simulink model "grid_nash"  (R2023b)
settings: Solver=ode23s  StartTime=0.0  StopTime=32  RelTol=1e-3
values from neighbouring files (symbols this model uses):
  lambda_compensator = -0.01    [model_parameters.m]
  nbus = 6    [model_parameters.m]
  Ts = 5e-6    (= 5e-06)    [model_parameters.m]
undefined symbols (not defined in the file or in its folder): AG, gcbh, Grid, IBR, L, SG, sps_rtmsupport, TX
libraries: spsThreePhaseVIMeasurementLib x13, spsFourierLib x13, spsPowerPositiveSequenceLib x13, spsThreePhaseSeriesRLCBranchLib x10, spsThreePhaseSeriesRLCLoadLib x10, spsThreePhaseTransformerTwoWindingsLib x10, spsDCVoltageSourceLib x8, spsFirstOrderFilterLib x8, spsabctodq0Lib x8, spsSimplifiedSynchronousMachinepuUnitsLib x6, spsGroundLib x4, spsUniversalBridgeLib x4
(part 1 of 2)
settings Model: SimulationMode=rapid-accelerator  Creator=psernatorre  LastModifiedBy=psernatorre
settings DataIOCC: InitialState=initial_data_nash.xFinal  LoadInitialState=on  SaveFinalState=on  SaveOperatingPoint=on
settings GRTTargetCC: RTWCAPISignals=on  RTWCAPIParams=on

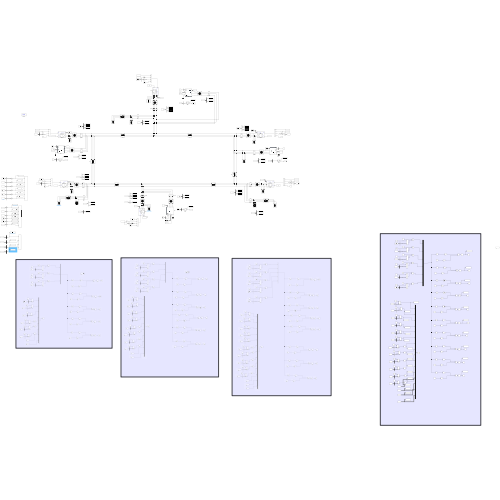
[thumbnail: Simulink's stored preview of the top-level diagram]
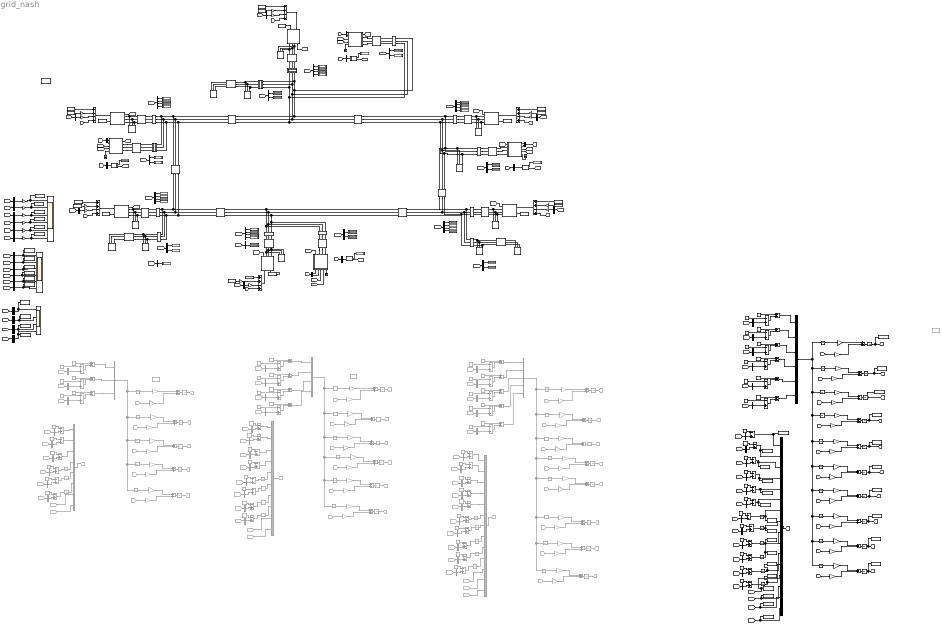
== system grid_nash ==
  note: NCG
  note: NCG
  note: NCG
  note: NCG
  Add{,6..7,20..22} (6 alike) : Sum  Inputs=++-+
  Add{1,3,14,23,25,27} (6 alike) : Sum  Inputs=+-
  Add{4..5,10,15,19,29..32,106} (10 alike) : Sum
  Add{39,44,51,56,61,68,73,78,83,90,95,100} (12 alike) : Sum  Commented=on  Inputs=+-
  Add{41..43,46..48,50,54..55,58..60,63..65,67,71..72,74..76,80..82,85..87,89,93..94,96..98,101..103} (36 alike) : Sum  Commented=on  Inputs=-+
  Add{40,45,49,52..53,57,62,66,69..70,77,79,84,88,91..92,99,104..105} (19 alike) : Sum  Commented=on
  Add{2,8..9,11..13,16..18,24,26,28,33..38} (18 alike) : Sum  Inputs=-+
  B1_IBR1 : Subsystem  mask{Sbase=Grid.Sbase, Vbase=Grid.Vbase, f=Grid.f, Ts=Ts, label=B1_IBR1, enable_power_calc=on}
      mask prompts: Sbase "Sbase (3-phase VA)"; Vbase "Vbase (L-L Vrms)"; f "Frequency (Hz)"; Ts "Sample time (s)"; label "Measure label"; enable_power_calc "Enable power calculation"
      mask init:
      | set_param([gcb '/signal'],'GotoTag', label)
      mask DialogControl DescGroupVar Prompt: Bus and measurements
      mask DialogControl Bus Prompt: Measure voltage, magnitude and phase, active power, reactive power
  B1_SG1 : Subsystem  mask{Sbase=Grid.Sbase, Vbase=Grid.Vbase, f=Grid.f, Ts=Ts, label=B1_SG1, enable_power_calc=on}
      mask prompts: Sbase "Sbase (3-phase VA)"; Vbase "Vbase (L-L Vrms)"; f "Frequency (Hz)"; Ts "Sample time (s)"; label "Measure label"; enable_power_calc "Enable power calculation"
      mask init:
      | set_param([gcb '/signal'],'GotoTag', label)
      mask DialogControl DescGroupVar Prompt: Bus and measurements
      mask DialogControl Bus Prompt: Measure voltage, magnitude and phase, active power, reactive power
  B5_L : Subsystem  mask{Sbase=Grid.Sbase, Vbase=Grid.Vbase, f=Grid.f, Ts=Ts, label=B5_L, enable_power_calc=on}
      mask prompts: Sbase "Sbase (3-phase VA)"; Vbase "Vbase (L-L Vrms)"; f "Frequency (Hz)"; Ts "Sample time (s)"; label "Measure label"; enable_power_calc "Enable power calculation"
      mask init:
      | set_param([gcb '/signal'],'GotoTag', label)
      mask DialogControl DescGroupVar Prompt: Bus and measurements
      mask DialogControl Bus Prompt: Measure voltage, magnitude and phase, active power, reactive power
  B5_SG6 : Subsystem  mask{Sbase=Grid.Sbase, Vbase=Grid.Vbase, f=Grid.f, Ts=Ts, label=B5_SG6, enable_power_calc=on}
      mask prompts: Sbase "Sbase (3-phase VA)"; Vbase "Vbase (L-L Vrms)"; f "Frequency (Hz)"; Ts "Sample time (s)"; label "Measure label"; enable_power_calc "Enable power calculation"
      mask init:
      | set_param([gcb '/signal'],'GotoTag', label)
      mask DialogControl DescGroupVar Prompt: Bus and measurements
      mask DialogControl Bus Prompt: Measure voltage, magnitude and phase, active power, reactive power
  B6_IBR3 : Subsystem  mask{Sbase=Grid.Sbase, Vbase=Grid.Vbase, f=Grid.f, Ts=Ts, label=B6_IBR3, enable_power_calc=on}
      mask prompts: Sbase "Sbase (3-phase VA)"; Vbase "Vbase (L-L Vrms)"; f "Frequency (Hz)"; Ts "Sample time (s)"; label "Measure label"; enable_power_calc "Enable power calculation"
      mask init:
      | set_param([gcb '/signal'],'GotoTag', label)
      mask DialogControl DescGroupVar Prompt: Bus and measurements
      mask DialogControl Bus Prompt: Measure voltage, magnitude and phase, active power, reactive power
  B6_SG5 : Subsystem  mask{Sbase=Grid.Sbase, Vbase=Grid.Vbase, f=Grid.f, Ts=Ts, label=B6_SG5, enable_power_calc=on}
      mask prompts: Sbase "Sbase (3-phase VA)"; Vbase "Vbase (L-L Vrms)"; f "Frequency (Hz)"; Ts "Sample time (s)"; label "Measure label"; enable_power_calc "Enable power calculation"
      mask init:
      | set_param([gcb '/signal'],'GotoTag', label)
      mask DialogControl DescGroupVar Prompt: Bus and measurements
      mask DialogControl Bus Prompt: Measure voltage, magnitude and phase, active power, reactive power
  B7_IBR4 : Subsystem  mask{Sbase=Grid.Sbase, Vbase=Grid.Vbase, f=Grid.f, Ts=Ts, label=B7_IBR4, enable_power_calc=on}
      mask prompts: Sbase "Sbase (3-phase VA)"; Vbase "Vbase (L-L Vrms)"; f "Frequency (Hz)"; Ts "Sample time (s)"; label "Measure label"; enable_power_calc "Enable power calculation"
      mask init:
      | set_param([gcb '/signal'],'GotoTag', label)
      mask DialogControl DescGroupVar Prompt: Bus and measurements
      mask DialogControl Bus Prompt: Measure voltage, magnitude and phase, active power, reactive power
  B7_L : Subsystem  mask{Sbase=Grid.Sbase, Vbase=Grid.Vbase, f=Grid.f, Ts=Ts, label=B7_L, enable_power_calc=on}
      mask prompts: Sbase "Sbase (3-phase VA)"; Vbase "Vbase (L-L Vrms)"; f "Frequency (Hz)"; Ts "Sample time (s)"; label "Measure label"; enable_power_calc "Enable power calculation"
      mask init:
      | set_param([gcb '/signal'],'GotoTag', label)
      mask DialogControl DescGroupVar Prompt: Bus and measurements
      mask DialogControl Bus Prompt: Measure voltage, magnitude and phase, active power, reactive power
  B7_SG4 : Subsystem  mask{Sbase=Grid.Sbase, Vbase=Grid.Vbase, f=Grid.f, Ts=Ts, label=B7_SG4, enable_power_calc=on}
      mask prompts: Sbase "Sbase (3-phase VA)"; Vbase "Vbase (L-L Vrms)"; f "Frequency (Hz)"; Ts "Sample time (s)"; label "Measure label"; enable_power_calc "Enable power calculation"
      mask init:
      | set_param([gcb '/signal'],'GotoTag', label)
      mask DialogControl DescGroupVar Prompt: Bus and measurements
      mask DialogControl Bus Prompt: Measure voltage, magnitude and phase, active power, reactive power
  B8_IBR2 : Subsystem  mask{Sbase=Grid.Sbase, Vbase=Grid.Vbase, f=Grid.f, Ts=Ts, label=B8_IBR2, enable_power_calc=on}
      mask prompts: Sbase "Sbase (3-phase VA)"; Vbase "Vbase (L-L Vrms)"; f "Frequency (Hz)"; Ts "Sample time (s)"; label "Measure label"; enable_power_calc "Enable power calculation"
      mask init:
      | set_param([gcb '/signal'],'GotoTag', label)
      mask DialogControl DescGroupVar Prompt: Bus and measurements
      mask DialogControl Bus Prompt: Measure voltage, magnitude and phase, active power, reactive power
  B8_SG3 : Subsystem  mask{Sbase=Grid.Sbase, Vbase=Grid.Vbase, f=Grid.f, Ts=Ts, label=B8_SG3, enable_power_calc=on}
      mask prompts: Sbase "Sbase (3-phase VA)"; Vbase "Vbase (L-L Vrms)"; f "Frequency (Hz)"; Ts "Sample time (s)"; label "Measure label"; enable_power_calc "Enable power calculation"
      mask init:
      | set_param([gcb '/signal'],'GotoTag', label)
      mask DialogControl DescGroupVar Prompt: Bus and measurements
      mask DialogControl Bus Prompt: Measure voltage, magnitude and phase, active power, reactive power
  B9_L : Subsystem  mask{Sbase=Grid.Sbase, Vbase=Grid.Vbase, f=Grid.f, Ts=Ts, label=B9_L, enable_power_calc=on}
      mask prompts: Sbase "Sbase (3-phase VA)"; Vbase "Vbase (L-L Vrms)"; f "Frequency (Hz)"; Ts "Sample time (s)"; label "Measure label"; enable_power_calc "Enable power calculation"
      mask init:
      | set_param([gcb '/signal'],'GotoTag', label)
      mask DialogControl DescGroupVar Prompt: Bus and measurements
      mask DialogControl Bus Prompt: Measure voltage, magnitude and phase, active power, reactive power
  B9_SG2 : Subsystem  mask{Sbase=Grid.Sbase, Vbase=Grid.Vbase, f=Grid.f, Ts=Ts, label=B9_SG2, enable_power_calc=on}
      mask prompts: Sbase "Sbase (3-phase VA)"; Vbase "Vbase (L-L Vrms)"; f "Frequency (Hz)"; Ts "Sample time (s)"; label "Measure label"; enable_power_calc "Enable power calculation"
      mask init:
      | set_param([gcb '/signal'],'GotoTag', label)
      mask DialogControl DescGroupVar Prompt: Bus and measurements
      mask DialogControl Bus Prompt: Measure voltage, magnitude and phase, active power, reactive power
  Bus Selector{1,29,31,33,91..92} (6 alike) : BusSelector  OutputSignals=P,Q,Vmag,Vphase
  Bus Selector{8,10..11,19,32,42..45,95} (10 alike) : BusSelector  OutputSignals=P
  Bus Selector{3..7,9,12..13,16..18,20..22,24..25,28,30,34,37,39..41,46..54} (32 alike) : BusSelector  OutputSignals=Rotor speed wm (pu)
  Bus Selector{14..15,35,93} (4 alike) : BusSelector  OutputSignals=V
  Bus Selector{2,23,26..27,36,38,94} (7 alike) : BusSelector  OutputSignals=P,Q
  Bus Selector{55..90} (36 alike) : BusSelector  Commented=on  OutputSignals=Rotor speed wm (pu)
  Constant{,17,20,23..24,28} (6 alike) : Constant  Value=1.02
  Constant1 : Constant  Value=0.20
  Constant{2,4,6..7,9..14,16,18..19,22,27,30,32,34,36..41} (24 alike) : Constant
  Constant15 : Constant  Value=0.10
  Constant21 : Constant  Value=0.05
  Constant25 : Constant  Value=0.50
  Constant26 : Constant  Value=0.40
  Constant29 : Constant  Value=0.05
  Constant{3,5,8,31,33,35} (6 alike) : Constant  Value=0
  Constant{42..46,48,50..51,53..58,60,62..63,65..66,68..74,76,78..79,81..82,84..86,88..89} (36 alike) : Constant  Commented=on
  Constant{47,49,52,59,61,64,67,75,77,80,83,87} (12 alike) : Constant  Commented=on  Value=0
  Demux{1..4} (4 alike) : Demux  Outputs=2
  Display{1..44} (44 alike) : Display
      settings: Format=bank
  From{84,88,92,100,104,108,117,121,125} (9 alike) : From  Commented=on  GotoTag=m_SG2
  From{85,91,93,101,107,109,118,124,126} (9 alike) : From  Commented=on  GotoTag=m_SG3
  From{83,86..87,99,102..103,119..120,136} (9 alike) : From  Commented=on  GotoTag=m_SG1
  From{81,89..90,94..95,97,105..106,110..111,116,122..123,127..128,133..134,141..142} (19 alike) : From  Commented=on
  From112 : From  Commented=on  GotoTag=m_IBR2
  From{113..115,130..132} (6 alike) : From  Commented=on  GotoTag=m_SG4
  From{6,12,24,26,34..35,70..72,150} (10 alike) : From
  From129 : From  Commented=on  GotoTag=m_IBR2
  From135 : From  Commented=on  GotoTag=m_IBR1
  From137 : From  Commented=on  GotoTag=m_SG5
  From138 : From  Commented=on  GotoTag=m_SG5
  From139 : From  Commented=on  GotoTag=m_SG5
  From140 : From  Commented=on  GotoTag=m_IBR3
  From82 : From  Commented=on  GotoTag=m_IBR1
  From96 : From  Commented=on  GotoTag=m_IBR2
  From98 : From  Commented=on  GotoTag=m_IBR1
  Gain{1,10..11,26..28} (6 alike) : Gain  Gain=Grid.f
  Gain12 : Gain  Gain=1/SG(4).Rp
  Gain13 : Gain  Gain=AG(4).Ki  Multiplication=Matrix(K*u)
  Gain14 : Gain  Gain=AG(4).Kp  Multiplication=Matrix(K*u)
  Gain15 : Gain  Gain=AG(5).Ki  Multiplication=Matrix(K*u)
  Gain16 : Gain  Gain=AG(5).Kp  Multiplication=Matrix(K*u)
  Gain17 : Gain  Gain=1/SG(2).Rp
  Gain18 : Gain  Gain=1/SG(2).Rp
  Gain19 : Gain  Gain=1/SG(3).Rp
  Gain2 : Gain  Gain=1/SG(1).Rp
  Gain20 : Gain  Gain=1/SG(3).Rp
  Gain21 : Gain  Gain=1/SG(4).Rp
  Gain22 : Gain  Gain=1/SG(5).Rp
  Gain23 : Gain  Gain=1/SG(5).Rp
  Gain24 : Gain  Gain=1/SG(6).Rp
  Gain25 : Gain  Gain=1/SG(6).Rp
  Gain29 : Gain  Gain=AG(6).Ki  Multiplication=Matrix(K*u)
  Gain3 : Gain  Gain=1/SG(1).Rp
  Gain30 : Gain  Gain=AG(6).Kp  Multiplication=Matrix(K*u)
  Gain31 : Gain  Gain=AG(7).Ki  Multiplication=Matrix(K*u)
  Gain32 : Gain  Gain=AG(7).Kp  Multiplication=Matrix(K*u)
  Gain33 : Gain  Gain=AG(8).Ki  Multiplication=Matrix(K*u)
  Gain34 : Gain  Gain=AG(8).Kp  Multiplication=Matrix(K*u)
  Gain35 : Gain  Gain=AG(9).Ki  Multiplication=Matrix(K*u)
  Gain36 : Gain  Gain=AG(9).Kp  Multiplication=Matrix(K*u)
  Gain37 : Gain  Commented=on  Gain=AG(4).Ki  Multiplication=Matrix(K*u)
  Gain38 : Gain  Commented=on  Gain=AG(4).Kp  Multiplication=Matrix(K*u)
  Gain39 : Gain  Commented=on  Gain=AG(5).Ki  Multiplication=Matrix(K*u)
  Gain4 : Gain  Gain=AG(1).Kp  Multiplication=Matrix(K*u)
  Gain40 : Gain  Commented=on  Gain=AG(5).Kp  Multiplication=Matrix(K*u)
  Gain41 : Gain  Commented=on  Gain=AG(1).Kp  Multiplication=Matrix(K*u)
  Gain42 : Gain  Commented=on  Gain=AG(1).Ki  Multiplication=Matrix(K*u)
  Gain43 : Gain  Commented=on  Gain=AG(2).Ki  Multiplication=Matrix(K*u)
  Gain44 : Gain  Commented=on  Gain=AG(2).Kp  Multiplication=Matrix(K*u)
  Gain45 : Gain  Commented=on  Gain=AG(3).Ki  Multiplication=Matrix(K*u)
  Gain46 : Gain  Commented=on  Gain=AG(3).Kp  Multiplication=Matrix(K*u)
  Gain47 : Gain  Commented=on  Gain=AG(5).Ki  Multiplication=Matrix(K*u)
  Gain48 : Gain  Commented=on  Gain=AG(5).Kp  Multiplication=Matrix(K*u)
  Gain49 : Gain  Commented=on  Gain=AG(6).Ki  Multiplication=Matrix(K*u)
  Gain5 : Gain  Gain=AG(1).Ki  Multiplication=Matrix(K*u)
  Gain50 : Gain  Commented=on  Gain=AG(6).Kp  Multiplication=Matrix(K*u)
  Gain51 : Gain  Commented=on  Gain=AG(1).Kp  Multiplication=Matrix(K*u)
  Gain52 : Gain  Commented=on  Gain=AG(1).Ki  Multiplication=Matrix(K*u)
  Gain53 : Gain  Commented=on  Gain=AG(2).Ki  Multiplication=Matrix(K*u)
  Gain54 : Gain  Commented=on  Gain=AG(2).Kp  Multiplication=Matrix(K*u)
  Gain55 : Gain  Commented=on  Gain=AG(3).Ki  Multiplication=Matrix(K*u)
  Gain56 : Gain  Commented=on  Gain=AG(3).Kp  Multiplication=Matrix(K*u)
  Gain57 : Gain  Commented=on  Gain=AG(4).Ki  Multiplication=Matrix(K*u)
  Gain58 : Gain  Commented=on  Gain=AG(4).Kp  Multiplication=Matrix(K*u)
  Gain59 : Gain  Commented=on  Gain=AG(6).Ki  Multiplication=Matrix(K*u)
  Gain6 : Gain  Gain=AG(2).Ki  Multiplication=Matrix(K*u)
  Gain60 : Gain  Commented=on  Gain=AG(6).Kp  Multiplication=Matrix(K*u)
  Gain61 : Gain  Commented=on  Gain=AG(7).Ki  Multiplication=Matrix(K*u)
  Gain62 : Gain  Commented=on  Gain=AG(7).Kp  Multiplication=Matrix(K*u)
  Gain63 : Gain  Commented=on  Gain=AG(1).Kp  Multiplication=Matrix(K*u)
  Gain64 : Gain  Commented=on  Gain=AG(1).Ki  Multiplication=Matrix(K*u)
  Gain65 : Gain  Commented=on  Gain=AG(2).Ki  Multiplication=Matrix(K*u)
  Gain66 : Gain  Commented=on  Gain=AG(2).Kp  Multiplication=Matrix(K*u)
  Gain67 : Gain  Commented=on  Gain=AG(3).Ki  Multiplication=Matrix(K*u)
  Gain68 : Gain  Commented=on  Gain=AG(3).Kp  Multiplication=Matrix(K*u)
  Gain69 : Gain  Commented=on  Gain=AG(4).Ki  Multiplication=Matrix(K*u)
  Gain7 : Gain  Gain=AG(2).Kp  Multiplication=Matrix(K*u)
  Gain70 : Gain  Commented=on  Gain=AG(4).Kp  Multiplication=Matrix(K*u)
  Gain71 : Gain  Commented=on  Gain=AG(5).Ki  Multiplication=Matrix(K*u)
  Gain72 : Gain  Commented=on  Gain=AG(5).Kp  Multiplication=Matrix(K*u)
  Gain73 : Gain  Commented=on  Gain=AG(8).Ki  Multiplication=Matrix(K*u)
  Gain74 : Gain  Commented=on  Gain=AG(8).Kp  Multiplication=Matrix(K*u)
  Gain75 : Gain  Gain=AG(10).Ki  Multiplication=Matrix(K*u)
  Gain76 : Gain  Gain=AG(10).Kp  Multiplication=Matrix(K*u)
  Gain8 : Gain  Gain=AG(3).Ki  Multiplication=Matrix(K*u)
  Gain9 : Gain  Gain=AG(3).Kp  Multiplication=Matrix(K*u)
  Goto2 : Goto
  Goto23 : Goto  Commented=on  GotoTag=u3
  Goto24 : Goto  Commented=on
  Goto25 : Goto  Commented=on  GotoTag=u7
  Goto26 : Goto  Commented=on  GotoTag=u8
  Goto27 : Goto  Commented=on  GotoTag=u1
  Goto28 : Goto  Commented=on  GotoTag=u2
  Goto29 : Goto  Commented=on  GotoTag=u3
  Goto30 : Goto  Commented=on
  Goto31 : Goto  Commented=on  GotoTag=u7
  Goto32 : Goto  Commented=on  GotoTag=u8
  Goto33 : Goto  Commented=on  GotoTag=u1
  Goto34 : Goto  Commented=on  GotoTag=u2
  Goto35 : Goto  Commented=on  GotoTag=u4
  Goto36 : Goto  Commented=on  GotoTag=u3
  Goto37 : Goto  Commented=on
  Goto38 : Goto  Commented=on  GotoTag=u7
  Goto39 : Goto  Commented=on  GotoTag=u8
  Goto40 : Goto  Commented=on  GotoTag=u1
  Goto41 : Goto  Commented=on  GotoTag=u2
  Goto42 : Goto  Commented=on  GotoTag=u4
  Goto43 : Goto  Commented=on  GotoTag=u5
  Goto44 : Goto  Commented=on  GotoTag=u9
  Ground{1..4} (4 alike) : spsGroundLib/Ground  LConnTagsString=a
  IBR1 : Subsystem  mask{S=Grid.Sbase, V=IBR(1).Vbase, Vdc=IBR(1).Vdc, Rf=IBR(1).Rf, Lf=IBR(1).Lf, Rc=IBR(1).Rc, Lc=IBR(1).Lc, Kp=IBR(1).Kp, Ki=IBR(1).Ki, f=Grid.f, Tf=IBR(1).Tf, Ts=Ts, enable_state_estimation=off, A_est=0, B_est=0, C_est=0, D_est=0}
      mask prompts: S "Pnom (VA)"; V "Vnom (Line Vrms)"; Vdc "Vdc (V)"; Rf "Rf (p.u.)"; Lf "Lf (p.u.)"; Rc "Rc (p.u.)"; Lc "Lc (p.u.)"; f "Frequency (Hz)"; Tf "Tf (feed-forward)"; Ts "Sample time (s)"; enable_state_estimation "Enable state estimation"
      mask DialogControl DescGroupVar Prompt: PLL-based grid-following IBR with LC filter
      mask DialogControl DescTextVar Prompt: Implements a grid-following inverter with LC filter with PI controllers in dq0-synchronous frames. It considers feed-forward compensation with first-order low-pass filter. Rf and Lf are impendances of the internal filter, and Rc and Lc are the impendances including a step-up transformer if there exists.
      mask Display: image('GFL_LC.png');
  IBR2 : Subsystem  mask{S=Grid.Sbase, V=IBR(2).Vbase, Vdc=IBR(2).Vdc, Rf=IBR(2).Rf, Lf=IBR(2).Lf, Rc=IBR(2).Rc, Lc=IBR(2).Lc, Kp=IBR(2).Kp, Ki=IBR(2).Ki, f=Grid.f, Tf=IBR(2).Tf, Ts=Ts, enable_state_estimation=off, A_est=0, B_est=0, C_est=0, D_est=0}
      mask prompts: S "Pnom (VA)"; V "Vnom (Line Vrms)"; Vdc "Vdc (V)"; Rf "Rf (p.u.)"; Lf "Lf (p.u.)"; Rc "Rc (p.u.)"; Lc "Lc (p.u.)"; f "Frequency (Hz)"; Tf "Tf (feed-forward)"; Ts "Sample time (s)"; enable_state_estimation "Enable state estimation"
      mask DialogControl DescGroupVar Prompt: PLL-based grid-following IBR with LC filter
      mask DialogControl DescTextVar Prompt: Implements a grid-following inverter with LC filter with PI controllers in dq0-synchronous frames. It considers feed-forward compensation with first-order low-pass filter. Rf and Lf are impendances of the internal filter, and Rc and Lc are the impendances including a step-up transformer if there exists.
      mask Display: image('GFL_LC.png');
  IBR3 : Subsystem  mask{S=Grid.Sbase, V=IBR(3).Vbase, Vdc=IBR(3).Vdc, Rf=IBR(3).Rf, Lf=IBR(3).Lf, Rc=IBR(3).Rc, Lc=IBR(3).Lc, Kp=IBR(3).Kp, Ki=IBR(3).Ki, f=Grid.f, Tf=IBR(3).Tf, Ts=Ts, enable_state_estimation=off, A_est=0, B_est=0, C_est=0, D_est=0}
      mask prompts: S "Pnom (VA)"; V "Vnom (Line Vrms)"; Vdc "Vdc (V)"; Rf "Rf (p.u.)"; Lf "Lf (p.u.)"; Rc "Rc (p.u.)"; Lc "Lc (p.u.)"; f "Frequency (Hz)"; Tf "Tf (feed-forward)"; Ts "Sample time (s)"; enable_state_estimation "Enable state estimation"
      mask DialogControl DescGroupVar Prompt: PLL-based grid-following IBR with LC filter
      mask DialogControl DescTextVar Prompt: Implements a grid-following inverter with LC filter with PI controllers in dq0-synchronous frames. It considers feed-forward compensation with first-order low-pass filter. Rf and Lf are impendances of the internal filter, and Rc and Lc are the impendances including a step-up transformer if there exists.
      mask Display: image('GFL_LC.png');
  IBR4 : Subsystem  mask{S=Grid.Sbase, V=IBR(2).Vbase, Vdc=IBR(2).Vdc, Rf=IBR(2).Rf, Lf=IBR(2).Lf, Rc=IBR(2).Rc, Lc=IBR(2).Lc, Kp=IBR(2).Kp, Ki=IBR(2).Ki, f=Grid.f, Tf=IBR(2).Tf, Ts=Ts, enable_state_estimation=off, A_est=0, B_est=0, C_est=0, D_est=0}
      mask prompts: S "Pnom (VA)"; V "Vnom (Line Vrms)"; Vdc "Vdc (V)"; Rf "Rf (p.u.)"; Lf "Lf (p.u.)"; Rc "Rc (p.u.)"; Lc "Lc (p.u.)"; f "Frequency (Hz)"; Tf "Tf (feed-forward)"; Ts "Sample time (s)"; enable_state_estimation "Enable state estimation"
      mask DialogControl DescGroupVar Prompt: PLL-based grid-following IBR with LC filter
      mask DialogControl DescTextVar Prompt: Implements a grid-following inverter with LC filter with PI controllers in dq0-synchronous frames. It considers feed-forward compensation with first-order low-pass filter. Rf and Lf are impendances of the internal filter, and Rc and Lc are the impendances including a step-up transformer if there exists.
      mask Display: image('GFL_LC.png');
  Integrator{,1..14,46} (16 alike) : Integrator
  Integrator{15..45} (31 alike) : Integrator  Commented=on
  Mux : Mux  Inputs=6
  Mux1 : Mux  Commented=on  Inputs=3
  Mux2 : Mux  Commented=on  Inputs=8
  Mux3 : Mux  Commented=on
  Mux4 : Mux  Commented=on  Inputs=10
  Mux5 : Mux  Commented=on  Inputs=5
  Mux6 : Mux  Inputs=16
  Mux7 : Mux  Commented=on  Inputs=13
  PLL (3ph) : Subsystem  AncestorBlock=|  DialogController=POWERSYS.PowerSysDialog  LoadFcn=sps_rtmsupport('LoadFcn', gcbh);  StartFcn=sps_rtmsupport('StartFcn', gcbh);  StopFcn=sps_rtmsupport('StopFcn', gcbh);  mask(PLL (3ph)){Fmin=45, Par_Init=[0, 60], ParK=[180, 3200, 1], TcD=1e-4, MaxRateChangeFreq=12, FilterCutOffFreq=25, Ts=Ts, AGC=on}
      | sps_lib/Control/PLL
      | (3ph)
      mask prompts: Fmin "Minimum frequency (Hz):"; Par_Init "Initial inputs [ Phase (degrees), Frequency (Hz) ]:"; ParK "Regulator gains [ Kp, Ki, Kd ]:"; TcD "Time constant for derivative action (s):"; MaxRateChangeFreq "Maximum rate of change of frequency (Hz/s):"; FilterCutOffFreq "Filter cut-off frequency for frequency measurement (Hz):"; Ts "Sample time:"; AGC "Enable automatic gain control"
      mask help:
      | This Phase Locked Loop (PLL) system can be used  to synchronize on a set of variable frequency, three-phase sinusoidal signals. If the Automatic Gain Control is enabled, the input (phase error) of the PLL regulator is scaled according to the input signals magnitude.
      |
      | For optimal performance, set regulator gains [ Kp Ki  Kd ] = [ 180  3200  1 ] and check the Enable Automatic Gain Control parameter.
      |
      | Input : Vector containing the normalized three-phase signals [Va Vb Vc]
      | Output 1:  Measured frequency (Hz) = w/(2pi)
      | Output 2:  Ramp w.t varying between  0 and 2*pi, synchronized on zero crossings of the fundamental (positive-sequence) of phase A.
      mask init:
      | block=gcb;
      | [WantBlockChoice,Ts,sps] = powericon('PLL3phInit',block,Fmin,Par_Init,ParK,TcD, MaxRateChangeFreq, FilterCutOffFreq, AGC,Ts);
      | powericon('SetInternalModels','set',block,WantBlockChoice);
      settings: CopyFcn=sps_rtmsupport('CopyFcn', gcbh);  DeleteFcn=sps_rtmsupport('DeleteFcn', gcbh);  UndoDeleteFcn=sps_rtmsupport('UndoDeleteFcn', gcbh);  ModelCloseFcn=sps_rtmsupport('ModelCloseFcn', gcbh);  PreSaveFcn=sps_rtmsupport('PreSaveFcn', gcbh);  PostSaveFcn=sps_rtmsupport('PostSaveFcn', gcbh);  NameChangeFcn=sps_rtmsupport('NameChangeFcn', gcbh);  PreCopyFcn=sps_rtmsupport('PreCopyFcn', gcbh);  OpenFcn=sps_rtmsupport('OpenFcn', gcbh, [8]);  CloseFcn=sps_rtmsupport('CloseFcn', gcbh);  PreDeleteFcn=sps_rtmsupport('PreDeleteFcn', gcbh);
      settings: LibrarySourceBlock=|
      | sps_lib/Control/PLL
      | (3ph)
      mask Help: helpview(psbhelp);
  PLL (3ph)1 : Subsystem  AncestorBlock=|  DialogController=POWERSYS.PowerSysDialog  LoadFcn=sps_rtmsupport('LoadFcn', gcbh);  StartFcn=sps_rtmsupport('StartFcn', gcbh);  StopFcn=sps_rtmsupport('StopFcn', gcbh);  mask(PLL (3ph)){Fmin=45, Par_Init=[0, 60], ParK=[180, 3200, 1], TcD=1e-4, MaxRateChangeFreq=12, FilterCutOffFreq=25, Ts=Ts, AGC=on}
      | sps_lib/Control/PLL
      | (3ph)
      mask prompts: Fmin "Minimum frequency (Hz):"; Par_Init "Initial inputs [ Phase (degrees), Frequency (Hz) ]:"; ParK "Regulator gains [ Kp, Ki, Kd ]:"; TcD "Time constant for derivative action (s):"; MaxRateChangeFreq "Maximum rate of change of frequency (Hz/s):"; FilterCutOffFreq "Filter cut-off frequency for frequency measurement (Hz):"; Ts "Sample time:"; AGC "Enable automatic gain control"
      mask help:
      | This Phase Locked Loop (PLL) system can be used  to synchronize on a set of variable frequency, three-phase sinusoidal signals. If the Automatic Gain Control is enabled, the input (phase error) of the PLL regulator is scaled according to the input signals magnitude.
      |
      | For optimal performance, set regulator gains [ Kp Ki  Kd ] = [ 180  3200  1 ] and check the Enable Automatic Gain Control parameter.
      |
      | Input : Vector containing the normalized three-phase signals [Va Vb Vc]
      | Output 1:  Measured frequency (Hz) = w/(2pi)
      | Output 2:  Ramp w.t varying between  0 and 2*pi, synchronized on zero crossings of the fundamental (positive-sequence) of phase A.
      mask init:
      | block=gcb;
      | [WantBlockChoice,Ts,sps] = powericon('PLL3phInit',block,Fmin,Par_Init,ParK,TcD, MaxRateChangeFreq, FilterCutOffFreq, AGC,Ts);
      | powericon('SetInternalModels','set',block,WantBlockChoice);
      settings: CopyFcn=sps_rtmsupport('CopyFcn', gcbh);  DeleteFcn=sps_rtmsupport('DeleteFcn', gcbh);  UndoDeleteFcn=sps_rtmsupport('UndoDeleteFcn', gcbh);  ModelCloseFcn=sps_rtmsupport('ModelCloseFcn', gcbh);  PreSaveFcn=sps_rtmsupport('PreSaveFcn', gcbh);  PostSaveFcn=sps_rtmsupport('PostSaveFcn', gcbh);  NameChangeFcn=sps_rtmsupport('NameChangeFcn', gcbh);  PreCopyFcn=sps_rtmsupport('PreCopyFcn', gcbh);  OpenFcn=sps_rtmsupport('OpenFcn', gcbh, [8]);  CloseFcn=sps_rtmsupport('CloseFcn', gcbh);  PreDeleteFcn=sps_rtmsupport('PreDeleteFcn', gcbh);
      settings: LibrarySourceBlock=|
      | sps_lib/Control/PLL
      | (3ph)
      mask Help: helpview(psbhelp);
  PLL (3ph)2 : Subsystem  AncestorBlock=|  DialogController=POWERSYS.PowerSysDialog  LoadFcn=sps_rtmsupport('LoadFcn', gcbh);  StartFcn=sps_rtmsupport('StartFcn', gcbh);  StopFcn=sps_rtmsupport('StopFcn', gcbh);  mask(PLL (3ph)){Fmin=45, Par_Init=[0, 60], ParK=[180, 3200, 1], TcD=1e-4, MaxRateChangeFreq=12, FilterCutOffFreq=25, Ts=Ts, AGC=on}
      | sps_lib/Control/PLL
      | (3ph)
      mask prompts: Fmin "Minimum frequency (Hz):"; Par_Init "Initial inputs [ Phase (degrees), Frequency (Hz) ]:"; ParK "Regulator gains [ Kp, Ki, Kd ]:"; TcD "Time constant for derivative action (s):"; MaxRateChangeFreq "Maximum rate of change of frequency (Hz/s):"; FilterCutOffFreq "Filter cut-off frequency for frequency measurement (Hz):"; Ts "Sample time:"; AGC "Enable automatic gain control"
      mask help:
      | This Phase Locked Loop (PLL) system can be used  to synchronize on a set of variable frequency, three-phase sinusoidal signals. If the Automatic Gain Control is enabled, the input (phase error) of the PLL regulator is scaled according to the input signals magnitude.
      |
      | For optimal performance, set regulator gains [ Kp Ki  Kd ] = [ 180  3200  1 ] and check the Enable Automatic Gain Control parameter.
      |
      | Input : Vector containing the normalized three-phase signals [Va Vb Vc]
      | Output 1:  Measured frequency (Hz) = w/(2pi)
      | Output 2:  Ramp w.t varying between  0 and 2*pi, synchronized on zero crossings of the fundamental (positive-sequence) of phase A.
      mask init:
      | block=gcb;
      | [WantBlockChoice,Ts,sps] = powericon('PLL3phInit',block,Fmin,Par_Init,ParK,TcD, MaxRateChangeFreq, FilterCutOffFreq, AGC,Ts);
      | powericon('SetInternalModels','set',block,WantBlockChoice);
      settings: CopyFcn=sps_rtmsupport('CopyFcn', gcbh);  DeleteFcn=sps_rtmsupport('DeleteFcn', gcbh);  UndoDeleteFcn=sps_rtmsupport('UndoDeleteFcn', gcbh);  ModelCloseFcn=sps_rtmsupport('ModelCloseFcn', gcbh);  PreSaveFcn=sps_rtmsupport('PreSaveFcn', gcbh);  PostSaveFcn=sps_rtmsupport('PostSaveFcn', gcbh);  NameChangeFcn=sps_rtmsupport('NameChangeFcn', gcbh);  PreCopyFcn=sps_rtmsupport('PreCopyFcn', gcbh);  OpenFcn=sps_rtmsupport('OpenFcn', gcbh, [8]);  CloseFcn=sps_rtmsupport('CloseFcn', gcbh);  PreDeleteFcn=sps_rtmsupport('PreDeleteFcn', gcbh);
      settings: LibrarySourceBlock=|
      | sps_lib/Control/PLL
      | (3ph)
      mask Help: helpview(psbhelp);
  PLL (3ph)3 : Subsystem  AncestorBlock=|  DialogController=POWERSYS.PowerSysDialog  LoadFcn=sps_rtmsupport('LoadFcn', gcbh);  StartFcn=sps_rtmsupport('StartFcn', gcbh);  StopFcn=sps_rtmsupport('StopFcn', gcbh);  mask(PLL (3ph)){Fmin=45, Par_Init=[0, 60], ParK=[180, 3200, 1], TcD=1e-4, MaxRateChangeFreq=12, FilterCutOffFreq=25, Ts=Ts, AGC=on}
      | sps_lib/Control/PLL
      | (3ph)
      mask prompts: Fmin "Minimum frequency (Hz):"; Par_Init "Initial inputs [ Phase (degrees), Frequency (Hz) ]:"; ParK "Regulator gains [ Kp, Ki, Kd ]:"; TcD "Time constant for derivative action (s):"; MaxRateChangeFreq "Maximum rate of change of frequency (Hz/s):"; FilterCutOffFreq "Filter cut-off frequency for frequency measurement (Hz):"; Ts "Sample time:"; AGC "Enable automatic gain control"
      mask help:
      | This Phase Locked Loop (PLL) system can be used  to synchronize on a set of variable frequency, three-phase sinusoidal signals. If the Automatic Gain Control is enabled, the input (phase error) of the PLL regulator is scaled according to the input signals magnitude.
      |
      | For optimal performance, set regulator gains [ Kp Ki  Kd ] = [ 180  3200  1 ] and check the Enable Automatic Gain Control parameter.
      |
      | Input : Vector containing the normalized three-phase signals [Va Vb Vc]
      | Output 1:  Measured frequency (Hz) = w/(2pi)
      | Output 2:  Ramp w.t varying between  0 and 2*pi, synchronized on zero crossings of the fundamental (positive-sequence) of phase A.
      mask init:
      | block=gcb;
      | [WantBlockChoice,Ts,sps] = powericon('PLL3phInit',block,Fmin,Par_Init,ParK,TcD, MaxRateChangeFreq, FilterCutOffFreq, AGC,Ts);
      | powericon('SetInternalModels','set',block,WantBlockChoice);
      settings: CopyFcn=sps_rtmsupport('CopyFcn', gcbh);  DeleteFcn=sps_rtmsupport('DeleteFcn', gcbh);  UndoDeleteFcn=sps_rtmsupport('UndoDeleteFcn', gcbh);  ModelCloseFcn=sps_rtmsupport('ModelCloseFcn', gcbh);  PreSaveFcn=sps_rtmsupport('PreSaveFcn', gcbh);  PostSaveFcn=sps_rtmsupport('PostSaveFcn', gcbh);  NameChangeFcn=sps_rtmsupport('NameChangeFcn', gcbh);  PreCopyFcn=sps_rtmsupport('PreCopyFcn', gcbh);  OpenFcn=sps_rtmsupport('OpenFcn', gcbh, [8]);  CloseFcn=sps_rtmsupport('CloseFcn', gcbh);  PreDeleteFcn=sps_rtmsupport('PreDeleteFcn', gcbh);
      settings: LibrarySourceBlock=|
      | sps_lib/Control/PLL
      | (3ph)
      mask Help: helpview(psbhelp);
  SG1 : spsSimplifiedSynchronousMachinepuUnitsLib/Simplified Synchronous Machine pu Units  ConnectionType=3-wire Y  MechanicalLoad=Mechanical power Pm  MeasurementBus=off  NominalParameters=[SG(1).Sbase SG(1).Vbase Grid.f]  Mechanical=[SG(1).H SG(1).KD 20]  InternalRL="[0.02  0.3]"  InitialConditions=[0 6.93594 0.40802 0.40802 0.40802 0.604989 -119.395 120.605]  IterativeDiscreteModel=Trapezoidal non iterative  TsBlock=-1  TsPowergui=0  LoadFlowParameters=[1,0,0,0,0]  Units=0  BusType=swing  Pref=20000000  Qref=0  Qmin=-Inf  Qmax=Inf  PLF=0  QLF=0
      settings: LibrarySourceBlock=|
      | sps_lib/Electrical Machines/Simplified Synchronous
      | Machine pu Units
  SG2 : spsSimplifiedSynchronousMachinepuUnitsLib/Simplified Synchronous Machine pu Units  ConnectionType=3-wire Y  MechanicalLoad=Mechanical power Pm  MeasurementBus=off  NominalParameters=[SG(2).Sbase SG(2).Vbase Grid.f]  Mechanical=[SG(2).H SG(2).KD 20]  InternalRL="[0.02  0.3]"  InitialConditions=[0 1.16591 0.202284 0.202284 0.202284 -10.8065 -130.807 109.193]  IterativeDiscreteModel=Trapezoidal non iterative  TsBlock=-1  TsPowergui=0  LoadFlowParameters=[1,0,0,0,0]  Units=0  BusType=PV  Pref=20000000  Qref=0  Qmin=-Inf  Qmax=Inf  PLF=0  QLF=0
      settings: LibrarySourceBlock=|
      | sps_lib/Electrical Machines/Simplified Synchronous
      | Machine pu Units
  SG3 : spsSimplifiedSynchronousMachinepuUnitsLib/Simplified Synchronous Machine pu Units  ConnectionType=3-wire Y  MechanicalLoad=Mechanical power Pm  MeasurementBus=off  NominalParameters=[SG(3).Sbase SG(3).Vbase Grid.f]  Mechanical=[SG(3).H SG(3).KD 20]  InternalRL="[0.02  0.3]"  InitialConditions=[0 2.15966 0.200038 0.200038 0.200038 -0.157653 -120.158 119.842]  IterativeDiscreteModel=Trapezoidal non iterative  TsBlock=-1  TsPowergui=0  LoadFlowParameters=[1,0,0,0,0]  Units=0  BusType=PV  Pref=20000000  Qref=0  Qmin=-Inf  Qmax=Inf  PLF=0  QLF=0
      settings: LibrarySourceBlock=|
      | sps_lib/Electrical Machines/Simplified Synchronous
      | Machine pu Units
  SG4 : spsSimplifiedSynchronousMachinepuUnitsLib/Simplified Synchronous Machine pu Units  ConnectionType=3-wire Y  MechanicalLoad=Mechanical power Pm  MeasurementBus=off  NominalParameters=[SG(4).Sbase SG(4).Vbase Grid.f]  Mechanical=[SG(4).H SG(4).KD 20]  InternalRL="[0.02  0.3]"  InitialConditions=[0 -3.45004 0.102056 0.102056 0.102056 -16.653 -136.653 103.347]  IterativeDiscreteModel=Trapezoidal non iterative  TsBlock=-1  TsPowergui=0  LoadFlowParameters=[1,0,0,0,0]  Units=0  BusType=PV  Pref=10000000  Qref=0  Qmin=-Inf  Qmax=Inf  PLF=0  QLF=0
      settings: LibrarySourceBlock=|
      | sps_lib/Electrical Machines/Simplified Synchronous
      | Machine pu Units
  SG5 : spsSimplifiedSynchronousMachinepuUnitsLib/Simplified Synchronous Machine pu Units  ConnectionType=3-wire Y  MechanicalLoad=Mechanical power Pm  MeasurementBus=off  NominalParameters=[SG(5).Sbase SG(5).Vbase Grid.f]  Mechanical=[SG(5).H SG(5).KD 20]  InternalRL="[0.02  0.3]"  InitialConditions=[0 -3.45004 0.102056 0.102056 0.102056 -16.653 -136.653 103.347]  IterativeDiscreteModel=Trapezoidal non iterative  TsBlock=-1  TsPowergui=0  LoadFlowParameters=[1,0,0,0,0]  Units=0  BusType=PV  Pref=10000000  Qref=0  Qmin=-Inf  Qmax=Inf  PLF=0  QLF=0
      settings: LibrarySourceBlock=|
      | sps_lib/Electrical Machines/Simplified Synchronous
      | Machine pu Units
  SG6 : spsSimplifiedSynchronousMachinepuUnitsLib/Simplified Synchronous Machine pu Units  ConnectionType=3-wire Y  MechanicalLoad=Mechanical power Pm  MeasurementBus=off  NominalParameters=[SG(6).Sbase SG(6).Vbase Grid.f]  Mechanical=[SG(6).H SG(6).KD 20]  InternalRL="[0.02  0.3]"  InitialConditions=[0 -3.45004 0.102056 0.102056 0.102056 -16.653 -136.653 103.347]  IterativeDiscreteModel=Trapezoidal non iterative  TsBlock=-1  TsPowergui=0  LoadFlowParameters=[1,0,0,0,0]  Units=0  BusType=PV  Pref=10000000  Qref=0  Qmin=-Inf  Qmax=Inf  PLF=0  QLF=0
      settings: LibrarySourceBlock=|
      | sps_lib/Electrical Machines/Simplified Synchronous
      | Machine pu Units
  Scope : Scope  NumInputPorts=6
  Scope1 : Scope  NumInputPorts=6
  Scope2 : Scope  NumInputPorts=4
  State-Space1 : StateSpace  Commented=on  A=lambda_compensator*eye(nbus)  B=eye(nbus)  C=eye(nbus)  D=zeros(nbus,nbus)  InitialCondition=0
  State-Space2 : StateSpace  Commented=on  A=lambda_compensator*eye(nbus)  B=eye(nbus)  C=eye(nbus)  D=zeros(nbus,nbus)  InitialCondition=0
  State-Space3 : StateSpace  Commented=on  A=lambda_compensator*eye(nbus)  B=eye(nbus)  C=eye(nbus)  D=zeros(nbus,nbus)  InitialCondition=0
  TX1 : spsThreePhaseSeriesRLCBranchLib/Three-Phase Series RLC Branch  LConnTagsString=A|B|C  RConnTagsString=A|B|C  BranchType=RL  Resistance=TX(1).R_ohm  Inductance=TX(1).L_H  Capacitance=1e-6  Measurements=None
  TX2 : spsThreePhaseSeriesRLCBranchLib/Three-Phase Series RLC Branch  LConnTagsString=A|B|C  RConnTagsString=A|B|C  BranchType=RL  Resistance=TX(2).R_ohm  Inductance=TX(2).L_H  Capacitance=1e-6  Measurements=None
  TX3 : spsThreePhaseSeriesRLCBranchLib/Three-Phase Series RLC Branch  LConnTagsString=A|B|C  RConnTagsString=A|B|C  BranchType=RL  Resistance=TX(3).R_ohm  Inductance=TX(3).L_H  Capacitance=1e-6  Measurements=None
  TX4 : spsThreePhaseSeriesRLCBranchLib/Three-Phase Series RLC Branch  LConnTagsString=A|B|C  RConnTagsString=A|B|C  BranchType=RL  Resistance=TX(4).R_ohm  Inductance=TX(4).L_H  Capacitance=1e-6  Measurements=None
  TX5 : spsThreePhaseSeriesRLCBranchLib/Three-Phase Series RLC Branch  LConnTagsString=A|B|C  RConnTagsString=A|B|C  BranchType=RL  Resistance=TX(5).R_ohm  Inductance=TX(5).L_H  Capacitance=1e-6  Measurements=None
  TX6 : spsThreePhaseSeriesRLCBranchLib/Three-Phase Series RLC Branch  LConnTagsString=A|B|C  RConnTagsString=A|B|C  BranchType=RL  Resistance=TX(6).R_ohm  Inductance=TX(6).L_H  Capacitance=1e-6  Measurements=None
  Three-Phase Parallel RLC Load : spsThreePhaseParallelRLCLoadLib/Three-Phase Parallel RLC Load  LConnTagsString=A|B|C  Configuration=Y (grounded)  NominalVoltage=Grid.Vbase  Vabc=[1e3 1e3 1e3]  Vabcp=[1e3 1e3 1e3]  NominalFrequency=60  UnbalancedPower=off  ActivePower=L(5).P  InductivePower=0  CapacitivePower=L(5).QC  Pabc=[10e3 9e3 11e3]  QLabc=[100 90 110]  QCabc=[100 90 110]  Pabcp=[10e3 9e3 11e3]  QLabcp=[100 90 110]  QCabcp=[100 90 110]  Measurements=None  LoadType=constant Z
  Three-Phase Parallel RLC Load1 : spsThreePhaseParallelRLCLoadLib/Three-Phase Parallel RLC Load  LConnTagsString=A|B|C  Configuration=Y (grounded)  NominalVoltage=(229163)*1.00253  Vabc=[1e3 1e3 1e3]  Vabcp=[1e3 1e3 1e3]  NominalFrequency=60  UnbalancedPower=off  ActivePower=20000000  InductivePower=0  CapacitivePower=0  Pabc=[10e3 9e3 11e3]  QLabc=[100 90 110]  QCabc=[100 90 110]  Pabcp=[10e3 9e3 11e3]  QLabcp=[100 90 110]  QCabcp=[100 90 110]  Measurements=None  LoadType=constant Z
  Three-Phase Parallel RLC Load2 : spsThreePhaseParallelRLCLoadLib/Three-Phase Parallel RLC Load  LConnTagsString=A|B|C  Configuration=Y (grounded)  NominalVoltage=Grid.Vbase  Vabc=[1e3 1e3 1e3]  Vabcp=[1e3 1e3 1e3]  NominalFrequency=60  UnbalancedPower=off  ActivePower=L(1).P  InductivePower=0  CapacitivePower=L(1).QC  Pabc=[10e3 9e3 11e3]  QLabc=[100 90 110]  QCabc=[100 90 110]  Pabcp=[10e3 9e3 11e3]  QLabcp=[100 90 110]  QCabcp=[100 90 110]  Measurements=None  LoadType=constant Z
  Three-Phase Series RLC Load1 : spsThreePhaseSeriesRLCLoadLib/Three-Phase Series RLC Load  LConnTagsString=A|B|C  Configuration=Y (grounded)  NominalVoltage=Grid.Vbase  Vabc=[1e3 1e3 1e3]  Vabcp=[1e3 1e3 1e3]  NominalFrequency=Grid.f  UnbalancedPower=off  ActivePower=L(2).P*1  InductivePower=0  CapacitivePower=0  Pabc=[10e3 9e3 11e3]  QLabc=[100 90 110]  QCabc=[100 90 110]  Pabcp=[10e3 9e3 11e3]  QLabcp=[100 90 110]  QCabcp=[100 90 110]  Measurements=None  LoadType=constant Z
  Three-Phase Series RLC Load10 : spsThreePhaseSeriesRLCLoadLib/Three-Phase Series RLC Load  LConnTagsString=A|B|C  Configuration=Y (grounded)  NominalVoltage=Grid.Vbase  Vabc=[1e3 1e3 1e3]  Vabcp=[1e3 1e3 1e3]  NominalFrequency=Grid.f  UnbalancedPower=off  ActivePower=L(6).P  InductivePower=0  CapacitivePower=0  Pabc=[10e3 9e3 11e3]  QLabc=[100 90 110]  QCabc=[100 90 110]  Pabcp=[10e3 9e3 11e3]  QLabcp=[100 90 110]  QCabcp=[100 90 110]  Measurements=None  LoadType=constant Z
  Three-Phase Series RLC Load11 : spsThreePhaseSeriesRLCLoadLib/Three-Phase Series RLC Load  LConnTagsString=A|B|C  Configuration=Y (grounded)  NominalVoltage=SG(2).Vbase  Vabc=[1e3 1e3 1e3]  Vabcp=[1e3 1e3 1e3]  NominalFrequency=Grid.f  UnbalancedPower=off  ActivePower=10000000  InductivePower=0  CapacitivePower=0  Pabc=[10e3 9e3 11e3]  QLabc=[100 90 110]  QCabc=[100 90 110]  Pabcp=[10e3 9e3 11e3]  QLabcp=[100 90 110]  QCabcp=[100 90 110]  Measurements=None  LoadType=constant Z
  Three-Phase Series RLC Load2 : spsThreePhaseSeriesRLCLoadLib/Three-Phase Series RLC Load  LConnTagsString=A|B|C  Configuration=Y (grounded)  NominalVoltage=SG(1).Vbase  Vabc=[1e3 1e3 1e3]  Vabcp=[1e3 1e3 1e3]  NominalFrequency=Grid.f  UnbalancedPower=off  ActivePower=20000000  InductivePower=0  CapacitivePower=0  Pabc=[10e3 9e3 11e3]  QLabc=[100 90 110]  QCabc=[100 90 110]  Pabcp=[10e3 9e3 11e3]  QLabcp=[100 90 110]  QCabcp=[100 90 110]  Measurements=None  LoadType=constant Z
  Three-Phase Series RLC Load3 : spsThreePhaseSeriesRLCLoadLib/Three-Phase Series RLC Load  LConnTagsString=A|B|C  Configuration=Y (grounded)  NominalVoltage=(229163)*1.00253  Vabc=[1e3 1e3 1e3]  Vabcp=[1e3 1e3 1e3]  NominalFrequency=Grid.f  UnbalancedPower=off  ActivePower=L(3).P  InductivePower=0  CapacitivePower=0  Pabc=[10e3 9e3 11e3]  QLabc=[100 90 110]  QCabc=[100 90 110]  Pabcp=[10e3 9e3 11e3]  QLabcp=[100 90 110]  QCabcp=[100 90 110]  Measurements=None  LoadType=constant PQ
  Three-Phase Series RLC Load4 : spsThreePhaseSeriesRLCLoadLib/Three-Phase Series RLC Load  LConnTagsString=A|B|C  Configuration=Y (grounded)  NominalVoltage=SG(2).Vbase  Vabc=[1e3 1e3 1e3]  Vabcp=[1e3 1e3 1e3]  NominalFrequency=Grid.f  UnbalancedPower=off  ActivePower=5000000  InductivePower=0  CapacitivePower=0  Pabc=[10e3 9e3 11e3]  QLabc=[100 90 110]  QCabc=[100 90 110]  Pabcp=[10e3 9e3 11e3]  QLabcp=[100 90 110]  QCabcp=[100 90 110]  Measurements=None  LoadType=constant Z
  Three-Phase Series RLC Load5 : spsThreePhaseSeriesRLCLoadLib/Three-Phase Series RLC Load  LConnTagsString=A|B|C  Configuration=Y (grounded)  NominalVoltage=SG(2).Vbase  Vabc=[1e3 1e3 1e3]  Vabcp=[1e3 1e3 1e3]  NominalFrequency=Grid.f  UnbalancedPower=off  ActivePower=10000000  InductivePower=0  CapacitivePower=0  Pabc=[10e3 9e3 11e3]  QLabc=[100 90 110]  QCabc=[100 90 110]  Pabcp=[10e3 9e3 11e3]  QLabcp=[100 90 110]  QCabcp=[100 90 110]  Measurements=None  LoadType=constant Z
  Three-Phase Series RLC Load6 : spsThreePhaseSeriesRLCLoadLib/Three-Phase Series RLC Load  LConnTagsString=A|B|C  Configuration=Y (grounded)  NominalVoltage=Grid.Vbase  Vabc=[1e3 1e3 1e3]  Vabcp=[1e3 1e3 1e3]  NominalFrequency=Grid.f  UnbalancedPower=off  ActivePower=L(2).P*2  InductivePower=0  CapacitivePower=0  Pabc=[10e3 9e3 11e3]  QLabc=[100 90 110]  QCabc=[100 90 110]  Pabcp=[10e3 9e3 11e3]  QLabcp=[100 90 110]  QCabcp=[100 90 110]  Measurements=None  LoadType=constant Z
  Three-Phase Series RLC Load7 : spsThreePhaseSeriesRLCLoadLib/Three-Phase Series RLC Load  LConnTagsString=A|B|C  Configuration=Y (grounded)  NominalVoltage=SG(2).Vbase  Vabc=[1e3 1e3 1e3]  Vabcp=[1e3 1e3 1e3]  NominalFrequency=Grid.f  UnbalancedPower=off  ActivePower=10000000  InductivePower=0  CapacitivePower=0  Pabc=[10e3 9e3 11e3]  QLabc=[100 90 110]  QCabc=[100 90 110]  Pabcp=[10e3 9e3 11e3]  QLabcp=[100 90 110]  QCabcp=[100 90 110]  Measurements=None  LoadType=constant Z
  Three-Phase Series RLC Load8 : spsThreePhaseSeriesRLCLoadLib/Three-Phase Series RLC Load  LConnTagsString=A|B|C  Configuration=Y (grounded)  NominalVoltage=SG(2).Vbase  Vabc=[1e3 1e3 1e3]  Vabcp=[1e3 1e3 1e3]  NominalFrequency=Grid.f  UnbalancedPower=off  ActivePower=5000000  InductivePower=0  CapacitivePower=0  Pabc=[10e3 9e3 11e3]  QLabc=[100 90 110]  QCabc=[100 90 110]  Pabcp=[10e3 9e3 11e3]  QLabcp=[100 90 110]  QCabcp=[100 90 110]  Measurements=None  LoadType=constant Z
  Three-Phase Transformer (Two Windings)1 : spsThreePhaseTransformerTwoWindingsLib/Three-Phase Transformer (Two Windings)  Winding1Connection=Yg  Winding2Connection=Yg  CoreType=Three single-phase transformers  SetSaturation=off  Hysteresis=off  DataFile='hysteresis'  SetInitialFlux=off  Measurements=None  UNITS=pu  NominalPower=[SG(1).TXR.Snom , Grid.f ]  Winding1=[ SG(1).Vbase , SG(1).TXR.R1 , SG(1).TXR.L1 ]  Winding2=[ Grid.Vbase , SG(1).TXR.R2 , SG(1).TXR.L2 ]  Rm=500  Lm=500  L0=2.866  Saturation=[ 0,0 ; 0.0024,1.2 ; 1.0,1.52 ]  InitialFluxes=[1273.5 -1273.5 1114.3]  BreakLoop=off  DiscreteSolver=Trapezoidal iterative  DataType=off  TransfoNumber=1
  Three-Phase Transformer (Two Windings)10 : spsThreePhaseTransformerTwoWindingsLib/Three-Phase Transformer (Two Windings)  Winding1Connection=Yg  Winding2Connection=Yg  CoreType=Three single-phase transformers  SetSaturation=off  Hysteresis=off  DataFile='hysteresis'  SetInitialFlux=off  Measurements=None  UNITS=pu  NominalPower=[IBR(2).TXR.Snom , Grid.f ]  Winding1=[ IBR(2).Vbase , IBR(2).TXR.R1 , IBR(2).TXR.L1 ]  Winding2=[ Grid.Vbase , IBR(2).TXR.R2 , IBR(2).TXR.L2 ]  Rm=600  Lm=500  L0=2.866  Saturation=[ 0,0 ; 0.0024,1.2 ; 1.0,1.52 ]  InitialFluxes=[1273.5 -1273.5 1114.3]  BreakLoop=off  DiscreteSolver=Trapezoidal iterative  DataType=off  TransfoNumber=1
  Three-Phase Transformer (Two Windings)2 : spsThreePhaseTransformerTwoWindingsLib/Three-Phase Transformer (Two Windings)  Winding1Connection=Yg  Winding2Connection=Yg  CoreType=Three single-phase transformers  SetSaturation=off  Hysteresis=off  DataFile='hysteresis'  SetInitialFlux=off  Measurements=None  UNITS=pu  NominalPower=[IBR(1).TXR.Snom , Grid.f ]  Winding1=[ IBR(1).Vbase , IBR(1).TXR.R1 , IBR(1).TXR.L1 ]  Winding2=[ Grid.Vbase , IBR(1).TXR.R2 , IBR(1).TXR.L2 ]  Rm=600  Lm=500  L0=2.866  Saturation=[ 0,0 ; 0.0024,1.2 ; 1.0,1.52 ]  InitialFluxes=[1273.5 -1273.5 1114.3]  BreakLoop=off  DiscreteSolver=Trapezoidal iterative  DataType=off  TransfoNumber=1
  Three-Phase Transformer (Two Windings)3 : spsThreePhaseTransformerTwoWindingsLib/Three-Phase Transformer (Two Windings)  Winding1Connection=Yg  Winding2Connection=Yg  CoreType=Three single-phase transformers  SetSaturation=off  Hysteresis=off  DataFile='hysteresis'  SetInitialFlux=off  Measurements=None  UNITS=pu  NominalPower=[SG(4).TXR.Snom , Grid.f ]  Winding1=[ SG(4).Vbase , SG(4).TXR.R1 , SG(4).TXR.L1 ]  Winding2=[ Grid.Vbase , SG(4).TXR.R2 , SG(4).TXR.L2 ]  Rm=500  Lm=500  L0=2.866  Saturation=[ 0,0 ; 0.0024,1.2 ; 1.0,1.52 ]  InitialFluxes=[1273.5 -1273.5 1114.3]  BreakLoop=off  DiscreteSolver=Trapezoidal iterative  DataType=off  TransfoNumber=1
  Three-Phase Transformer (Two Windings)4 : spsThreePhaseTransformerTwoWindingsLib/Three-Phase Transformer (Two Windings)  Winding1Connection=Yg  Winding2Connection=Yg  CoreType=Three single-phase transformers  SetSaturation=off  Hysteresis=off  DataFile='hysteresis'  SetInitialFlux=off  Measurements=None  UNITS=pu  NominalPower=[SG(5).TXR.Snom , Grid.f ]  Winding1=[ SG(5).Vbase , SG(5).TXR.R1 , SG(5).TXR.L1 ]  Winding2=[ Grid.Vbase , SG(5).TXR.R2 , SG(5).TXR.L2 ]  Rm=500  Lm=500  L0=2.866  Saturation=[ 0,0 ; 0.0024,1.2 ; 1.0,1.52 ]  InitialFluxes=[1273.5 -1273.5 1114.3]  BreakLoop=off  DiscreteSolver=Trapezoidal iterative  DataType=off  TransfoNumber=1
  Three-Phase Transformer (Two Windings)5 : spsThreePhaseTransformerTwoWindingsLib/Three-Phase Transformer (Two Windings)  Winding1Connection=Yg  Winding2Connection=Yg  CoreType=Three single-phase transformers  SetSaturation=off  Hysteresis=off  DataFile='hysteresis'  SetInitialFlux=off  Measurements=None  UNITS=pu  NominalPower=[IBR(2).TXR.Snom , Grid.f ]  Winding1=[ IBR(2).Vbase , IBR(2).TXR.R1 , IBR(2).TXR.L1 ]  Winding2=[ Grid.Vbase , IBR(2).TXR.R2 , IBR(2).TXR.L2 ]  Rm=600  Lm=500  L0=2.866  Saturation=[ 0,0 ; 0.0024,1.2 ; 1.0,1.52 ]  InitialFluxes=[1273.5 -1273.5 1114.3]  BreakLoop=off  DiscreteSolver=Trapezoidal iterative  DataType=off  TransfoNumber=1
  Three-Phase Transformer (Two Windings)6 : spsThreePhaseTransformerTwoWindingsLib/Three-Phase Transformer (Two Windings)  Winding1Connection=Yg  Winding2Connection=Yg  CoreType=Three single-phase transformers  SetSaturation=off  Hysteresis=off  DataFile='hysteresis'  SetInitialFlux=off  Measurements=None  UNITS=pu  NominalPower=[SG(2).TXR.Snom , Grid.f ]  Winding1=[ SG(2).Vbase , SG(2).TXR.R1 , SG(2).TXR.L1 ]  Winding2=[ Grid.Vbase , SG(2).TXR.R2 , SG(2).TXR.L2 ]  Rm=500  Lm=500  L0=2.866  Saturation=[ 0,0 ; 0.0024,1.2 ; 1.0,1.52 ]  InitialFluxes=[1273.5 -1273.5 1114.3]  BreakLoop=off  DiscreteSolver=Trapezoidal iterative  DataType=off  TransfoNumber=1
  Three-Phase Transformer (Two Windings)7 : spsThreePhaseTransformerTwoWindingsLib/Three-Phase Transformer (Two Windings)  Winding1Connection=Yg  Winding2Connection=Yg  CoreType=Three single-phase transformers  SetSaturation=off  Hysteresis=off  DataFile='hysteresis'  SetInitialFlux=off  Measurements=None  UNITS=pu  NominalPower=[SG(2).TXR.Snom , Grid.f ]  Winding1=[ SG(2).Vbase , SG(2).TXR.R1 , SG(2).TXR.L1 ]  Winding2=[ Grid.Vbase , SG(2).TXR.R2 , SG(2).TXR.L2 ]  Rm=500  Lm=500  L0=2.866  Saturation=[ 0,0 ; 0.0024,1.2 ; 1.0,1.52 ]  InitialFluxes=[1273.5 -1273.5 1114.3]  BreakLoop=off  DiscreteSolver=Trapezoidal iterative  DataType=off  TransfoNumber=1
  Three-Phase Transformer (Two Windings)8 : spsThreePhaseTransformerTwoWindingsLib/Three-Phase Transformer (Two Windings)  Winding1Connection=Yg  Winding2Connection=Yg  CoreType=Three single-phase transformers  SetSaturation=off  Hysteresis=off  DataFile='hysteresis'  SetInitialFlux=off  Measurements=None  UNITS=pu  NominalPower=[IBR(3).TXR.Snom , Grid.f ]  Winding1=[ IBR(3).Vbase , IBR(3).TXR.R1 , IBR(3).TXR.L1 ]  Winding2=[ Grid.Vbase , IBR(3).TXR.R2 , IBR(3).TXR.L2 ]  Rm=500  Lm=500  L0=2.866  Saturation=[ 0,0 ; 0.0024,1.2 ; 1.0,1.52 ]  InitialFluxes=[1273.5 -1273.5 1114.3]  BreakLoop=off  DiscreteSolver=Trapezoidal iterative  DataType=off  TransfoNumber=1
  Three-Phase Transformer (Two Windings)9 : spsThreePhaseTransformerTwoWindingsLib/Three-Phase Transformer (Two Windings)  Winding1Connection=Yg  Winding2Connection=Yg  CoreType=Three single-phase transformers  SetSaturation=off  Hysteresis=off  DataFile='hysteresis'  SetInitialFlux=off  Measurements=None  UNITS=pu  NominalPower=[SG(6).TXR.Snom , Grid.f ]  Winding1=[ SG(6).Vbase , SG(6).TXR.R1 , SG(6).TXR.L1 ]  Winding2=[ Grid.Vbase , SG(6).TXR.R2 , SG(6).TXR.L2 ]  Rm=500  Lm=500  L0=2.866  Saturation=[ 0,0 ; 0.0024,1.2 ; 1.0,1.52 ]  InitialFluxes=[1273.5 -1273.5 1114.3]  BreakLoop=off  DiscreteSolver=Trapezoidal iterative  DataType=off  TransfoNumber=1
  Three-Phase Breaker : spsThreePhaseBreakerLib/Three-Phase Breaker  InitialState=open  SwitchA=on  SwitchB=on  SwitchC=on  SwitchTimes=[13]  External=off  BreakerResistance=0.01  SnubberResistance=1e6  SnubberCapacitance=inf  Measurements=None
  Three-Phase Breaker1 : spsThreePhaseBreakerLib/Three-Phase Breaker  InitialState=open  SwitchA=on  SwitchB=on  SwitchC=on  SwitchTimes=[13 23]  External=off  BreakerResistance=0.01  SnubberResistance=1e6  SnubberCapacitance=inf  Measurements=None
  Three-Phase Breaker2 : spsThreePhaseBreakerLib/Three-Phase Breaker  InitialState=open  SwitchA=on  SwitchB=on  SwitchC=on  SwitchTimes=[40]  External=off  BreakerResistance=0.01  SnubberResistance=1e6  SnubberCapacitance=inf  Measurements=None
  To Workspace : ToWorkspace  VariableName=SG1_f  SaveFormat=Timeseries  SampleTime=10^(-4)
  To Workspace1 : ToWorkspace  VariableName=SG2_f  SaveFormat=Timeseries  SampleTime=10^(-4)
  To Workspace10 : ToWorkspace  VariableName=SG5_omega  SaveFormat=Timeseries  SampleTime=10^(-4)
  To Workspace11 : ToWorkspace  VariableName=delta1  SaveFormat=Timeseries  SampleTime=10^(-4)
  To Workspace12 : ToWorkspace  VariableName=SG6_omega  SaveFormat=Timeseries  SampleTime=10^(-4)
  To Workspace13 : ToWorkspace  VariableName=delta2  SaveFormat=Timeseries  SampleTime=10^(-4)
  To Workspace14 : ToWorkspace  VariableName=delta3  SaveFormat=Timeseries  SampleTime=10^(-4)
  To Workspace15 : ToWorkspace  VariableName=delta4  SaveFormat=Timeseries  SampleTime=10^(-4)
  To Workspace16 : ToWorkspace  VariableName=delta5  SaveFormat=Timeseries  SampleTime=10^(-4)
  To Workspace17 : ToWorkspace  VariableName=delta6  SaveFormat=Timeseries  SampleTime=10^(-4)
  To Workspace18 : ToWorkspace  VariableName=x_IBR1  SaveFormat=Timeseries  SampleTime=10^(-4)
  To Workspace19 : ToWorkspace  VariableName=x_IBR2  SaveFormat=Timeseries  SampleTime=10^(-4)
  To Workspace2 : ToWorkspace  VariableName=SG3_f  SaveFormat=Timeseries  SampleTime=10^(-4)
  To Workspace20 : ToWorkspace  VariableName=x_IBR3  SaveFormat=Timeseries  SampleTime=10^(-4)
  To Workspace21 : ToWorkspace  VariableName=SG1_u  SaveFormat=Timeseries  SampleTime=10^(-4)
  To Workspace22 : ToWorkspace  VariableName=SG2_u  SaveFormat=Timeseries  SampleTime=10^(-4)
  To Workspace23 : ToWorkspace  VariableName=SG3_u  SaveFormat=Timeseries  SampleTime=10^(-4)
  To Workspace24 : ToWorkspace  VariableName=SG4_u  SaveFormat=Timeseries  SampleTime=10^(-4)
  To Workspace25 : ToWorkspace  VariableName=SG5_u  SaveFormat=Timeseries  SampleTime=10^(-4)
  To Workspace26 : ToWorkspace  VariableName=SG6_u  SaveFormat=Timeseries  SampleTime=10^(-4)
  To Workspace27 : ToWorkspace  VariableName=IBR1_u  SaveFormat=Timeseries  SampleTime=10^(-4)
  To Workspace28 : ToWorkspace  VariableName=IBR2_u  SaveFormat=Timeseries  SampleTime=10^(-4)
  To Workspace29 : ToWorkspace  VariableName=IBR3_u  SaveFormat=Timeseries  SampleTime=10^(-4)
  To Workspace3 : ToWorkspace  VariableName=SG4_f  SaveFormat=Timeseries  SampleTime=10^(-4)
  To Workspace30 : ToWorkspace  VariableName=IBR4_u  SaveFormat=Timeseries  SampleTime=10^(-4)
  To Workspace31 : ToWorkspace  VariableName=x_IBR4  SaveFormat=Timeseries  SampleTime=10^(-4)
  To Workspace32 : ToWorkspace  VariableName=SG1_p  SaveFormat=Timeseries  SampleTime=10^(-4)
  To Workspace33 : ToWorkspace  VariableName=SG2_p  SaveFormat=Timeseries  SampleTime=10^(-4)
  To Workspace34 : ToWorkspace  VariableName=SG3_p  SaveFormat=Timeseries  SampleTime=10^(-4)
  To Workspace35 : ToWorkspace  VariableName=SG4_p  SaveFormat=Timeseries  SampleTime=10^(-4)
  To Workspace36 : ToWorkspace  VariableName=SG5_p  SaveFormat=Timeseries  SampleTime=10^(-4)
  To Workspace37 : ToWorkspace  VariableName=SG6_p  SaveFormat=Timeseries  SampleTime=10^(-4)
  To Workspace38 : ToWorkspace  VariableName=IBR1_p  SaveFormat=Timeseries  SampleTime=10^(-4)
  To Workspace39 : ToWorkspace  VariableName=IBR2_p  SaveFormat=Timeseries  SampleTime=10^(-4)
  To Workspace4 : ToWorkspace  VariableName=SG5_f  SaveFormat=Timeseries  SampleTime=10^(-4)
  To Workspace40 : ToWorkspace  VariableName=IBR3_p  SaveFormat=Timeseries  SampleTime=10^(-4)
  To Workspace41 : ToWorkspace  VariableName=IBR4_p  SaveFormat=Timeseries  SampleTime=10^(-4)
  To Workspace5 : ToWorkspace  VariableName=SG6_f  SaveFormat=Timeseries  SampleTime=10^(-4)
  To Workspace6 : ToWorkspace  VariableName=SG1_omega  SaveFormat=Timeseries  SampleTime=10^(-4)
  To Workspace7 : ToWorkspace  VariableName=SG2_omega  SaveFormat=Timeseries  SampleTime=10^(-4)
  To Workspace8 : ToWorkspace  VariableName=SG3_omega  SaveFormat=Timeseries  SampleTime=10^(-4)
  To Workspace9 : ToWorkspace  VariableName=SG4_omega  SaveFormat=Timeseries  SampleTime=10^(-4)
  Unit Delay{1..9,29} (10 alike) : UnitDelay  SampleTime=Ts  HasFrameUpgradeWarning=on
  Unit Delay{10..28} (19 alike) : UnitDelay  Commented=on  SampleTime=Ts  HasFrameUpgradeWarning=on
  powergui : sps_lib/powergui  Priority=1  SimulationMode=Discrete  SampleTime=Ts  frequency=60  Iterations=50  frequencyindice=0  Pbase=100e6  ErrMax=1e-4  UnitsV=kV  UnitsW=MW  buscounter=0  FunctionMessages=off  echomessages=off  EnableUseOfTLC=off  CurrentSourceSwitches=off  DisableSnubberDevices=off  DisableRonSwitches=off  DisableVfSwitches=off  DisplayEquations=off  AutomaticDiscreteSolvers=off  SolverType=Tustin/Backward Euler (TBE)  Interpol=off  ExternalGateDelay=off  methode=off  Ts=100  x0status=blocks  SPID=on  SwTol=0  HookPort=off  NonlinearTolerance=1e-4  nMaxIteration=100  ContinueOnMaxIteration=off  RestoreLinks=warning  ResistiveCurrentMeasurement=off  Frange=[0:2:500]  Ylog=off  Xlog=on  ShowGrid=off  save=off  variable=ZData  structure=0  ZoomFFT=off  StartTime=0.0  cycles=1  DisplayStyle=1  fundamental=60  FreqAxis=off  MaxFrequency=1000  frequencyindicesteady=1  RmsSteady=1  display=off
  wires:
  Gain5/1 -> Add10/1
  From35/1 -> Gain7/1
  From12/1 -> Gain4/1
  Gain7/1 -> Add15/2
  Gain6/1 -> Add15/1
  Add10/1 -> Unit Delay1/1
  Add15/1 -> Unit Delay2/1
  Gain4/1 -> Add10/2
  Unit Delay1/1 -> To Workspace21/1, [u1]
  Unit Delay2/1 -> To Workspace22/1, [u2]
  Mux6/1 -> Goto2/1
  Constant8/1 -> Add1/1
  Bus Selector23/2 -> Display8/1  "<Q>"
  Bus Selector23/1 -> Display7/1  "<P>"
  [B8_IBR2] -> IBR2/3(Inport)
  Demux1/2 -> IBR2/2(In2)
  [B8_IBR2] -> Bus Selector23/1
  [B8_wt] -> IBR2/4(Inport1)
  IBR2/1(Outport) -> [m_IBR2]
  Demux1/1 -> IBR2/1(In1)
  PLL (3ph)/2(wt) -> [B8_wt]
  PLL (3ph)/1(Freq) -> Display6/1
  [B1_SG1] -> Bus Selector1/1
  Bus Selector1/1 -> Display1/1  "<P>"
  Bus Selector1/2 -> Display2/1  "<Q>"
  Bus Selector2/1 -> Display3/1  "<P>"
  Bus Selector2/2 -> Display4/1  "<Q>"
  [B9_L] -> Bus Selector2/1
  [m_SG1] -> Bus Selector3/1
  Bus Selector3/1 -> Display5/1  "<Rotor speed wm (pu)>"
  [m_SG1] -> Bus Selector7/1
  Bus Selector7/1 -> Gain1/1  "<Rotor speed wm (pu)>"
  [B1_SG1] -> Bus Selector10/1
  [B8_SG3] -> Bus Selector15/1
  Bus Selector15/1 -> PLL (3ph)/1(abc)  "<V>"
  [B1_IBR1] -> Bus Selector19/1
  Bus Selector1/3 -> Display9/1  "<Vmag>"
  Bus Selector1/4 -> Display10/1  "<Vphase>"
  Constant1/1 -> Add/1
  Bus Selector26/2 -> Display13/1  "<Q>"
  Bus Selector26/1 -> Display12/1  "<P>"
  [B1_IBR1] -> Bus Selector26/1
  Bus Selector6/1 -> Add2/2  "<Rotor speed wm (pu)>"
  Constant7/1 -> Add2/1
  [m_SG1] -> Bus Selector6/1
  Constant10/1 -> Add9/1
  [m_SG1] -> Bus Selector25/1
  Bus Selector25/1 -> Add9/2  "<Rotor speed wm (pu)>"
  Add9/1 -> Mux6/1, To Workspace6/1
  Add2/1 -> Add1/2
  Gain1/1 -> To Workspace/1, Scope/1
  Integrator7/1 -> Gain5/1
  Integrator6/1 -> Gain6/1
  Bus Selector24/1 -> Add11/2  "<Rotor speed wm (pu)>"
  [m_SG2] -> Bus Selector24/1
  Add11/1 -> To Workspace7/1, Mux6/2
  Constant13/1 -> Add11/1
  Bus Selector28/1 -> Add13/2  "<Rotor speed wm (pu)>"
  [m_SG3] -> Bus Selector28/1
  Constant16/1 -> Add13/1
  Add13/1 -> To Workspace8/1, Mux6/3
  Add1/1 -> Mux/1
  Add3/1 -> Mux/2
  From34/1 -> Gain9/1
  Integrator5/1 -> Gain8/1
  Gain9/1 -> Add19/2
  Gain8/1 -> Add19/1
  Add19/1 -> Unit Delay3/1
  Gain10/1 -> To Workspace1/1, Scope/2
  Bus Selector30/1 -> Gain10/1  "<Rotor speed wm (pu)>"
  [m_SG2] -> Bus Selector30/1
  [B8_IBR2] -> Bus Selector32/1
  Gain2/1 -> Add/3
  [m_SG1] -> Bus Selector4/1
  Bus Selector4/1 -> Gain2/1  "<Rotor speed wm (pu)>"
  Constant14/1 -> Gain3/1
  Gain3/1 -> Add/2
  Add4/1 -> Unit Delay4/1
  Unit Delay4/1 -> To Workspace24/1, [u4]
  Integrator4/1 -> Gain13/1
  Gain14/1 -> Add4/2
  From24/1 -> Gain14/1
  Gain13/1 -> Add4/1
  From26/1 -> Gain16/1
  Add5/1 -> Unit Delay5/1
  Integrator3/1 -> Gain15/1
  Gain15/1 -> Add5/1
  Gain16/1 -> Add5/2
  Unit Delay5/1 -> To Workspace25/1, [u5]
  Add/1 -> SG1/1
  Constant/1 -> SG1/2
  Gain17/1 -> Add6/3
  Gain18/1 -> Add6/2
  [m_SG2] -> Bus Selector9/1
  Constant19/1 -> Gain18/1
  Bus Selector9/1 -> Gain17/1  "<Rotor speed wm (pu)>"
  Constant21/1 -> Add6/1
  Add6/1 -> SG2/1
  Constant20/1 -> SG2/2
  SG2/1 -> [m_SG2]
  Gain19/1 -> Add7/3
  SG3/1 -> [m_SG3]
  Add7/1 -> SG3/1
  Constant22/1 -> Gain20/1
  Constant24/1 -> SG3/2
  Bus Selector12/1 -> Gain19/1  "<Rotor speed wm (pu)>"
  [m_SG3] -> Bus Selector12/1
  Constant25/1 -> Add7/1
  Gain20/1 -> Add7/2
  SG1/1 -> [m_SG1]
  Demux3/1 -> IBR1/1(In1)
  Demux3/2 -> IBR1/2(In2)
  IBR1/1(Outport) -> [m_IBR1]
  [u7] -> Demux3/1
  [B1_IBR1] -> IBR1/3(Inport)
  [B1_wt] -> IBR1/4(Inport1)
  [m_SG3] -> Bus Selector5/1
  Bus Selector5/1 -> Gain11/1  "<Rotor speed wm (pu)>"
  Gain11/1 -> To Workspace2/1, Scope/3
  [B9_SG2] -> Bus Selector8/1
  [B8_SG3] -> Bus Selector11/1
  PLL (3ph)1/1(Freq) -> Display11/1
  PLL (3ph)1/2(wt) -> [B1_wt]
  Bus Selector14/1 -> PLL (3ph)1/1(abc)  "<V>"
  [B1_SG1] -> Bus Selector14/1
  [m_SG2] -> Bus Selector16/1
  Bus Selector16/1 -> Add8/2  "<Rotor speed wm (pu)>"
  Constant2/1 -> Add8/1
  Add8/1 -> Add3/2
  Constant3/1 -> Add3/1
  Constant5/1 -> Add14/1
  Bus Selector17/1 -> Add16/2  "<Rotor speed wm (pu)>"
  Constant4/1 -> Add16/1
  [m_SG3] -> Bus Selector17/1
  Add16/1 -> Add14/2
  Add14/1 -> Mux/3
  SG4/1 -> [m_SG4]
  Bus Selector22/1 -> Gain12/1  "<Rotor speed wm (pu)>"
  Constant15/1 -> Add20/1
  Gain21/1 -> Add20/2
  Constant12/1 -> Gain21/1
  Gain12/1 -> Add20/3
  [m_SG4] -> Bus Selector22/1
  Add20/1 -> SG4/1
  Constant17/1 -> SG4/2
  Bus Selector27/1 -> Display14/1  "<P>"
  [B7_L] -> Bus Selector27/1
  Bus Selector27/2 -> Display15/1  "<Q>"
  Bus Selector29/2 -> Display18/1  "<Q>"
  Bus Selector29/4 -> Display17/1  "<Vphase>"
  [B8_SG3] -> Bus Selector29/1
  Bus Selector29/3 -> Display19/1  "<Vmag>"
  Bus Selector29/1 -> Display16/1  "<P>"
  Bus Selector31/1 -> Display20/1  "<P>"
  Bus Selector31/3 -> Display23/1  "<Vmag>"
  Bus Selector31/4 -> Display21/1  "<Vphase>"
  [B9_SG2] -> Bus Selector31/1
  Bus Selector31/2 -> Display22/1  "<Q>"
  Bus Selector33/1 -> Display24/1  "<P>"
  Bus Selector33/3 -> Display27/1  "<Vmag>"
  Bus Selector33/4 -> Display25/1  "<Vphase>"
  [B7_SG4] -> Bus Selector33/1
  Bus Selector33/2 -> Display26/1  "<Q>"
  Constant18/1 -> Gain23/1
  Gain23/1 -> Add21/2
  Constant26/1 -> Add21/1
  Bus Selector34/1 -> Gain22/1  "<Rotor speed wm (pu)>"
  Gain22/1 -> Add21/3
  [m_SG5] -> Bus Selector34/1
  SG5/1 -> [m_SG5]
  Constant23/1 -> SG5/2
  Add21/1 -> SG5/1
  [B6_IBR3] -> IBR3/3(Inport)
  Demux2/2 -> IBR3/2(In2)
  Demux2/1 -> IBR3/1(In1)
  Bus Selector36/2 -> Display30/1  "<Q>"
  [B6_IBR3] -> Bus Selector36/1
  IBR3/1(Outport) -> [m_IBR3]
  [B6_wt] -> IBR3/4(Inport1)
  PLL (3ph)2/2(wt) -> [B6_wt]
  PLL (3ph)2/1(Freq) -> Display28/1
  [B6_SG5] -> Bus Selector35/1
  Bus Selector36/1 -> Display29/1  "<P>"
  [m_SG6] -> Bus Selector37/1
  Constant27/1 -> Gain25/1
  Constant28/1 -> SG6/2
  Gain25/1 -> Add22/2
  Bus Selector37/1 -> Gain24/1  "<Rotor speed wm (pu)>"
  Add22/1 -> SG6/1
  Gain24/1 -> Add22/3
  Constant29/1 -> Add22/1
  SG6/1 -> [m_SG6]
  Bus Selector38/1 -> Display31/1  "<P>"
  [B5_L] -> Bus Selector38/1
  Bus Selector38/2 -> Display32/1  "<Q>"
  Bus Selector39/1 -> Gain26/1  "<Rotor speed wm (pu)>"
  [m_SG4] -> Bus Selector39/1
  Gain26/1 -> To Workspace3/1, Scope/4
  Bus Selector40/1 -> Gain27/1  "<Rotor speed wm (pu)>"
  Gain27/1 -> To Workspace4/1, Scope/5
  [m_SG5] -> Bus Selector40/1
  Gain28/1 -> To Workspace5/1, Scope/6
  Bus Selector41/1 -> Gain28/1  "<Rotor speed wm (pu)>"
  [m_SG6] -> Bus Selector41/1
  [B6_SG5] -> Bus Selector42/1
  Bus Selector10/1 -> To Workspace32/1, Scope1/1  "<P>"
  Bus Selector8/1 -> To Workspace33/1, Scope1/2  "<P>"
  Bus Selector11/1 -> To Workspace34/1, Scope1/3  "<P>"
  Bus Selector42/1 -> To Workspace36/1, Scope1/5  "<P>"
  Bus Selector43/1 -> To Workspace37/1, Scope1/6  "<P>"
  [B5_SG6] -> Bus Selector43/1
  Bus Selector44/1 -> To Workspace35/1, Scope1/4  "<P>"
  [B7_SG4] -> Bus Selector44/1
  Bus Selector19/1 -> To Workspace38/1, Scope2/1  "<P>"
  Bus Selector32/1 -> To Workspace39/1, Scope2/2  "<P>"
  Bus Selector45/1 -> To Workspace40/1, Scope2/3  "<P>"
  [B6_IBR3] -> Bus Selector45/1
  Constant30/1 -> Add24/1
  Bus Selector46/1 -> Add24/2  "<Rotor speed wm (pu)>"
  [m_SG4] -> Bus Selector46/1
  Add24/1 -> Add23/2
  Add23/1 -> Mux/4
  Constant31/1 -> Add23/1
  Bus Selector47/1 -> Add26/2  "<Rotor speed wm (pu)>"
  [m_SG5] -> Bus Selector47/1
  Constant33/1 -> Add25/1
  Add26/1 -> Add25/2
  Constant32/1 -> Add26/1
  Add28/1 -> Add27/2
  Constant34/1 -> Add28/1
  Constant35/1 -> Add27/1
  [m_SG6] -> Bus Selector48/1
  Bus Selector48/1 -> Add28/2  "<Rotor speed wm (pu)>"
  Add27/1 -> Mux/6
  From6/1 -> Gain30/1
  Integrator8/1 -> Gain29/1
  Gain29/1 -> Add29/1
  Gain30/1 -> Add29/2
  Unit Delay6/1 -> To Workspace26/1, [u6]
  Add29/1 -> Unit Delay6/1
  Unit Delay7/1 -> To Workspace27/1, [u7]
  Add30/1 -> Unit Delay7/1
  Gain31/1 -> Add30/1
  Integrator9/1 -> Gain31/1
  From70/1 -> Gain32/1
  Gain32/1 -> Add30/2
  Add31/1 -> Unit Delay8/1
  Integrator10/1 -> Gain33/1
  Gain34/1 -> Add31/2
  Unit Delay8/1 -> To Workspace28/1, [u8]
  Gain33/1 -> Add31/1
  From71/1 -> Gain34/1
  Gain35/1 -> Add32/1
  From72/1 -> Gain36/1
  Integrator11/1 -> Gain35/1
  Add32/1 -> Unit Delay9/1
  Gain36/1 -> Add32/2
  Unit Delay9/1 -> To Workspace29/1, [u9]
  Constant36/1 -> Add33/1
  Add33/1 -> To Workspace9/1, Mux6/4
  [m_SG4] -> Bus Selector13/1
  Bus Selector13/1 -> Add33/2  "<Rotor speed wm (pu)>"
  Bus Selector49/1 -> Add34/2  "<Rotor speed wm (pu)>"
  [m_SG5] -> Bus Selector49/1
  Constant37/1 -> Add34/1
  [m_SG6] -> Bus Selector50/1
  Constant38/1 -> Add35/1
  Bus Selector50/1 -> Add35/2  "<Rotor speed wm (pu)>"
  Bus Selector21/1 -> Add38/2  "<Rotor speed wm (pu)>"
  Constant6/1 -> Add38/1
  Bus Selector53/1 -> Add37/2  "<Rotor speed wm (pu)>"
  [m_SG3] -> Bus Selector51/1
  Bus Selector52/1 -> Add36/2  "<Rotor speed wm (pu)>"
  Constant40/1 -> Add36/1
  Bus Selector20/1 -> Add12/2  "<Rotor speed wm (pu)>"
  [m_SG5] -> Bus Selector52/1
  [m_SG1] -> Bus Selector21/1
  Add37/1 -> Integrator14/1
  Add18/1 -> Integrator12/1
  Constant39/1 -> Add18/1
  Add36/1 -> Integrator13/1
  [m_SG4] -> Bus Selector18/1
  [m_SG6] -> Bus Selector53/1
  Bus Selector18/1 -> Add18/2  "<Rotor speed wm (pu)>"
  Constant41/1 -> Add37/1
  Add38/1 -> Integrator/1
  [m_SG2] -> Bus Selector20/1
  Constant9/1 -> Add12/1
  Constant11/1 -> Add17/1
  Add17/1 -> Integrator2/1
  Bus Selector51/1 -> Add17/2  "<Rotor speed wm (pu)>"
  Add12/1 -> Integrator1/1
  Integrator/1 -> To Workspace11/1, Mux6/7
  [m_IBR1] -> To Workspace18/1, Mux6/13
  Integrator1/1 -> To Workspace13/1, Mux6/8
  Integrator2/1 -> Mux6/9, To Workspace14/1
  Integrator12/1 -> Mux6/10, To Workspace15/1
  [m_IBR2] -> To Workspace19/1, Mux6/14
  [m_IBR3] -> To Workspace20/1, Mux6/15
  [m_SG2] -> Bus Selector54/1
  Bus Selector54/1 -> Display33/1  "<Rotor speed wm (pu)>"
  Bus Selector35/1 -> PLL (3ph)2/1(abc)  "<V>"
  [u1] -> Add/4
  [u2] -> Add6/4
  [u8] -> Demux1/1
  [u3] -> Add7/4
  From86/1 -> Bus Selector58/1
  Add48/1 -> Integrator15/1
  Add43/1 -> Mux2/3
  Bus Selector62/1 -> Add43/2  "<Rotor speed wm (pu)>"
  Add50/1 -> Add39/2
  Constant49/1 -> Add44/1
  Add55/1 -> Mux2/1
  Add40/1 -> Unit Delay10/1
  Add41/1 -> Mux2/2
  Add53/1 -> Unit Delay14/1
  Constant53/1 -> Add42/1
  Gain43/1 -> Add45/1
  From88/1 -> Bus Selector60/1
  Add49/1 -> Unit Delay12/1
  Bus Selector56/1 -> Add46/2  "<Rotor speed wm (pu)>"
  Bus Selector59/1 -> Add47/2  "<Rotor speed wm (pu)>"
  From93/1 -> Bus Selector59/1
  Integrator17/1 -> Mux2/6
  From83/1 -> Bus Selector61/1
  Constant42/1 -> Add55/1
  Add42/1 -> Integrator16/1
  Add54/1 -> Add51/2
  Bus Selector63/1 -> Add50/2  "<Rotor speed wm (pu)>"
  Gain44/1 -> Add45/2
  Constant51/1 -> Add50/1
  From84/1 -> Bus Selector55/1
  Unit Delay14/1 -> Goto26/1
  Integrator19/1 -> Gain37/1
  From91/1 -> Bus Selector62/1
  Add46/1 -> Add44/2
  Integrator21/1 -> Gain43/1
  Integrator20/1 -> Gain45/1
  Add44/1 -> Mux1/3
  Gain40/1 -> Add53/2
  Unit Delay12/1 -> Goto23/1
  Constant50/1 -> Add48/1
  Constant45/1 -> Add43/1
  From92/1 -> Bus Selector57/1
  Add51/1 -> Mux1/2
  From82/1 -> Mux2/7
  Bus Selector58/1 -> Add48/2  "<Rotor speed wm (pu)>"
  Gain37/1 -> Add52/1
  Mux1/1 -> Integrator22/1, Integrator21/1, Integrator20/1, Integrator19/1, Integrator18/1
  Gain46/1 -> Add49/2
  Unit Delay13/1 -> Goto25/1
  From90/1 -> Gain40/1
  Bus Selector57/1 -> Add42/2  "<Rotor speed wm (pu)>"
  Add52/1 -> Unit Delay13/1
  Gain41/1 -> Add40/2
  Integrator18/1 -> Gain39/1
  Mux2/1 -> Goto24/1
  Bus Selector61/1 -> Add55/2  "<Rotor speed wm (pu)>"
  Constant44/1 -> Add41/1
  Gain45/1 -> Add49/1
  From87/1 -> Bus Selector63/1
  Gain38/1 -> Add52/2
  Bus Selector55/1 -> Add54/2  "<Rotor speed wm (pu)>"
  Gain39/1 -> Add53/1
  Add45/1 -> Unit Delay11/1
  Constant43/1 -> Add47/1
  Bus Selector60/1 -> Add41/2  "<Rotor speed wm (pu)>"
  Constant46/1 -> Add54/1
  From85/1 -> Bus Selector56/1
  Unit Delay10/1 -> Goto27/1
  Integrator15/1 -> Mux2/4
  From94/1 -> Gain46/1
  From81/1 -> Gain41/1
  Constant52/1 -> Add39/1
  Add39/1 -> Mux1/1
  From96/1 -> Mux2/8
  Unit Delay11/1 -> Goto28/1
  From95/1 -> Gain44/1
  From89/1 -> Gain38/1
  Constant48/1 -> Add46/1
  Constant47/1 -> Add51/1
  Integrator16/1 -> Mux2/5
  Add47/1 -> Integrator17/1
  Gain42/1 -> Add40/1
  Integrator22/1 -> Gain42/1
  Integrator13/1 -> To Workspace16/1, Mux6/11
  Integrator14/1 -> To Workspace17/1, Mux6/12
  Add34/1 -> To Workspace10/1, Mux6/5
  Add35/1 -> To Workspace12/1, Mux6/6
  Add25/1 -> Mux/5
  From102/1 -> Bus Selector67/1
  Add64/1 -> Integrator25/1
  Unit Delay18/1 -> Goto31/1
  Constant63/1 -> Add67/1
  Constant58/1 -> Add71/1
  From110/1 -> Gain56/1
  Add56/1 -> Mux3/1
  From98/1 -> Mux4/9
  Integrator26/1 -> Gain49/1
  Gain49/1 -> Add70/1
  Constant62/1 -> Add65/1
  Add72/1 -> Mux4/1
  Integrator25/1 -> Mux4/7
  Gain56/1 -> Add66/2
  From97/1 -> Gain51/1
  Constant61/1 -> Add61/1
  Integrator29/1 -> Gain53/1
  Add65/1 -> Integrator23/1
  From107/1 -> Bus Selector71/1
  Constant57/1 -> Add60/1
  From99/1 -> Bus Selector70/1
  Add62/1 -> Unit Delay16/1
  From100/1 -> Bus Selector64/1
  Bus Selector66/1 -> Add59/2  "<Rotor speed wm (pu)>"
  Integrator27/1 -> Gain47/1
  From104/1 -> Bus Selector69/1
  Unit Delay16/1 -> Goto34/1
  From112/1 -> Mux4/10
  Add59/1 -> Integrator24/1
  Bus Selector67/1 -> Add65/2  "<Rotor speed wm (pu)>"
  Unit Delay15/1 -> Goto33/1
  Integrator30/1 -> Gain52/1
  Bus Selector64/1 -> Add71/2  "<Rotor speed wm (pu)>"
  From109/1 -> Bus Selector68/1
  Mux4/1 -> Goto30/1
  Constant56/1 -> Add58/1
  Add70/1 -> Unit Delay19/1
  From101/1 -> Bus Selector65/1
  Gain55/1 -> Add66/1
  Integrator28/1 -> Gain55/1
  Constant65/1 -> Add59/1
  Add67/1 -> Add56/2
  Unit Delay19/1 -> Goto32/1
  Add61/1 -> Mux3/3
  Add69/1 -> Unit Delay18/1
  Constant54/1 -> Add72/1
  From111/1 -> Gain54/1
  Gain51/1 -> Add57/2
  Constant64/1 -> Add56/1
  Constant55/1 -> Add64/1
  From105/1 -> Gain48/1
  Unit Delay17/1 -> Goto29/1
  Constant59/1 -> Add68/1
  Gain52/1 -> Add57/1
  Bus Selector65/1 -> Add63/2  "<Rotor speed wm (pu)>"
  From108/1 -> Bus Selector66/1
  Gain53/1 -> Add62/1
  From106/1 -> Gain50/1
  Add71/1 -> Add68/2
  Add68/1 -> Mux3/2
  Gain54/1 -> Add62/2
  From103/1 -> Bus Selector72/1
  Add58/1 -> Mux4/2
  Bus Selector71/1 -> Add60/2  "<Rotor speed wm (pu)>"
  Bus Selector70/1 -> Add72/2  "<Rotor speed wm (pu)>"
  Add60/1 -> Mux4/3
  Bus Selector69/1 -> Add58/2  "<Rotor speed wm (pu)>"
  Bus Selector72/1 -> Add67/2  "<Rotor speed wm (pu)>"
  Gain50/1 -> Add70/2
  Integrator23/1 -> Mux4/5
  Integrator24/1 -> Mux4/6
  Add57/1 -> Unit Delay15/1
  Bus Selector68/1 -> Add64/2  "<Rotor speed wm (pu)>"
  Add66/1 -> Unit Delay17/1
  Gain48/1 -> Add69/2
  Constant60/1 -> Add63/1
  Add63/1 -> Add61/2
  Gain47/1 -> Add69/1
  Bus Selector73/1 -> Add74/2  "<Rotor speed wm (pu)>"
  Add74/1 -> Add73/2
  From113/1 -> Bus Selector73/1
  Constant67/1 -> Add73/1
  Constant66/1 -> Add74/1
  Add73/1 -> Mux3/4
  Add75/1 -> Mux4/4
  From114/1 -> Bus Selector74/1
  Bus Selector74/1 -> Add75/2  "<Rotor speed wm (pu)>"
  Constant68/1 -> Add75/1
  From115/1 -> Bus Selector75/1
  Constant69/1 -> Add76/1
  Bus Selector75/1 -> Add76/2  "<Rotor speed wm (pu)>"
  Add76/1 -> Integrator31/1
  Integrator31/1 -> Mux4/8
  Integrator32/1 -> Gain57/1
  Add77/1 -> Unit Delay20/1
  Unit Delay20/1 -> Goto35/1
  From116/1 -> Gain58/1
  Mux3/1 -> Integrator30/1, Integrator29/1, Integrator28/1, Integrator32/1, Integrator27/1, Integrator26/1
  Gain58/1 -> Add77/2
  Gain57/1 -> Add77/1
  [u4] -> Add20/4
  From119/1 -> Bus Selector79/1
  Bus Selector80/1 -> Add86/2  "<Rotor speed wm (pu)>"
  Unit Delay24/1 -> Goto38/1
  Mux7/1 -> Goto37/1
  Add93/1 -> Add90/2
  Unit Delay21/1 -> Goto40/1
  Constant82/1 -> Add96/1
  From126/1 -> Bus Selector80/1
  Add84/1 -> Unit Delay22/1
  From117/1 -> Bus Selector76/1
  Bus Selector87/1 -> Add98/2  "<Rotor speed wm (pu)>"
  Gain63/1 -> Add79/2
  Integrator37/1 -> Gain59/1
  From130/1 -> Bus Selector85/1
  Bus Selector84/1 -> Add89/2  "<Rotor speed wm (pu)>"
  From118/1 -> Bus Selector77/1
  From134/1 -> Gain63/1
  Unit Delay22/1 -> Goto41/1
  Add97/1 -> Mux7/4
  Add87/1 -> Integrator33/1
  Constant74/1 -> Add93/1
  Add89/1 -> Add78/2
  Constant72/1 -> Add80/1
  Add83/1 -> Mux5/3
  Constant85/1 -> Add98/1
  Integrator36/1 -> Gain61/1
  Add98/1 -> Integrator41/1
  Constant76/1 -> Add85/1
  Bus Selector86/1 -> Add97/2  "<Rotor speed wm (pu)>"
  Add99/1 -> Unit Delay26/1
  Add92/1 -> Unit Delay25/1
  Gain65/1 -> Add84/1
  Add78/1 -> Mux5/1
  From131/1 -> Bus Selector86/1
  Gain59/1 -> Add91/1
  Add86/1 -> Integrator35/1
  Constant83/1 -> Add95/1
  Constant80/1 -> Add78/1
  Integrator39/1 -> Gain65/1
  Bus Selector85/1 -> Add96/2  "<Rotor speed wm (pu)>"
  Constant84/1 -> Add97/1
  Constant79/1 -> Add89/1
  From133/1 -> Gain70/1
  Bus Selector83/1 -> Add82/2  "<Rotor speed wm (pu)>"
  Unit Delay26/1 -> Goto42/1
  Add79/1 -> Unit Delay21/1
  Constant73/1 -> Add82/1
  Add95/1 -> Mux5/4
  From136/1 -> Bus Selector82/1
  From120/1 -> Bus Selector84/1
  Gain70/1 -> Add99/2
  Bus Selector79/1 -> Add87/2  "<Rotor speed wm (pu)>"
  Constant71/1 -> Add86/1
  Constant81/1 -> Add81/1
  Bus Selector78/1 -> Add81/2  "<Rotor speed wm (pu)>"
  Gain66/1 -> Add84/2
  Add94/1 -> Mux7/1
  Bus Selector76/1 -> Add93/2  "<Rotor speed wm (pu)>"
  Gain69/1 -> Add99/1
  From123/1 -> Gain62/1
  Bus Selector81/1 -> Add80/2  "<Rotor speed wm (pu)>"
  Gain64/1 -> Add79/1
  Constant70/1 -> Add94/1
  Constant77/1 -> Add83/1
  Unit Delay25/1 -> Goto39/1
  Unit Delay23/1 -> Goto36/1
  Add82/1 -> Mux7/3
  Add91/1 -> Unit Delay24/1
  Integrator38/1 -> Gain67/1
  From132/1 -> Bus Selector87/1
  Bus Selector77/1 -> Add85/2  "<Rotor speed wm (pu)>"
  From122/1 -> Gain60/1
  From125/1 -> Bus Selector78/1
  Constant75/1 -> Add90/1
  Integrator40/1 -> Gain64/1
  Gain68/1 -> Add88/2
  Gain61/1 -> Add92/1
  Add90/1 -> Mux5/2
  Gain67/1 -> Add88/1
  From121/1 -> Bus Selector81/1
  Constant78/1 -> Add87/1
  From127/1 -> Gain68/1
  Integrator42/1 -> Gain69/1
  Add80/1 -> Mux7/2
  From128/1 -> Gain66/1
  Bus Selector82/1 -> Add94/2  "<Rotor speed wm (pu)>"
  Gain60/1 -> Add91/2
  From124/1 -> Bus Selector83/1
  Gain62/1 -> Add92/2
  Add85/1 -> Add83/2
  Add88/1 -> Unit Delay23/1
  Add96/1 -> Add95/2
  Add81/1 -> Integrator34/1
  From137/1 -> Bus Selector88/1
  Add100/1 -> Mux5/5
  Constant87/1 -> Add100/1
  Constant86/1 -> Add101/1
  Add101/1 -> Add100/2
  Bus Selector88/1 -> Add101/2  "<Rotor speed wm (pu)>"
  Constant88/1 -> Add102/1
  Bus Selector89/1 -> Add102/2  "<Rotor speed wm (pu)>"
  Add102/1 -> Mux7/5
  From138/1 -> Bus Selector89/1
  Integrator33/1 -> Mux7/6
  Integrator34/1 -> Mux7/7
  Integrator35/1 -> Mux7/8
  Integrator41/1 -> Mux7/9
  From139/1 -> Bus Selector90/1
  Bus Selector90/1 -> Add103/2  "<Rotor speed wm (pu)>"
  Add103/1 -> Integrator43/1
  Constant89/1 -> Add103/1
  Integrator43/1 -> Mux7/10
  From135/1 -> Mux7/11
  From129/1 -> Mux7/12
  From140/1 -> Mux7/13
  Gain71/1 -> Add104/1
  Integrator44/1 -> Gain71/1
  Add104/1 -> Unit Delay27/1
  Unit Delay27/1 -> Goto43/1
  From141/1 -> Gain72/1
  Gain72/1 -> Add104/2
  From142/1 -> Gain74/1
  Integrator45/1 -> Gain73/1
  Unit Delay28/1 -> Goto44/1
  Gain74/1 -> Add105/2
  Add105/1 -> Unit Delay28/1
  Gain73/1 -> Add105/1
  Mux5/1 -> Integrator40/1, Integrator39/1, Integrator38/1, Integrator42/1, Integrator44/1, Integrator37/1, Integrator45/1, Integrator36/1
  Bus Selector91/3 -> Display37/1  "<Vmag>"
  Bus Selector91/4 -> Display35/1  "<Vphase>"
  Bus Selector91/1 -> Display34/1  "<P>"
  Bus Selector91/2 -> Display36/1  "<Q>"
  [B6_SG5] -> Bus Selector91/1
  [u9] -> Demux2/1
  [u5] -> Add21/4
  [u6] -> Add22/4
  Bus Selector92/3 -> Display41/1  "<Vmag>"
  Bus Selector92/4 -> Display39/1  "<Vphase>"
  Bus Selector92/1 -> Display38/1  "<P>"
  Bus Selector92/2 -> Display40/1  "<Q>"
  [B5_SG6] -> Bus Selector92/1
  Unit Delay3/1 -> To Workspace23/1, [u3]
  IBR4/1(Outport) -> [m_IBR4]
  Bus Selector94/1 -> Display43/1  "<P>"
  Demux4/1 -> IBR4/1(In1)
  PLL (3ph)3/2(wt) -> [B7_wt]
  [B7_SG4] -> Bus Selector93/1
  [B7_IBR4] -> IBR4/3(Inport)
  [B7_wt] -> IBR4/4(Inport1)
  PLL (3ph)3/1(Freq) -> Display42/1
  [u10] -> Demux4/1
  Bus Selector94/2 -> Display44/1  "<Q>"
  Bus Selector93/1 -> PLL (3ph)3/1(abc)  "<V>"
  Demux4/2 -> IBR4/2(In2)
  [B7_IBR4] -> Bus Selector94/1
  Gain76/1 -> Add106/2
  Add106/1 -> Unit Delay29/1
  Unit Delay29/1 -> To Workspace30/1, [u10]
  Gain75/1 -> Add106/1
  Integrator46/1 -> Gain75/1
  From150/1 -> Gain76/1
  Mux/1 -> Integrator7/1, Integrator6/1, Integrator5/1, Integrator4/1, Integrator46/1, Integrator11/1, Integrator10/1, Integrator9/1, Integrator8/1, Integrator3/1
  [m_IBR4] -> To Workspace31/1, Mux6/16
  [B7_IBR4] -> Bus Selector95/1
  Bus Selector95/1 -> Scope2/4, To Workspace41/1  "<P>"
  connections:
  Three-Phase Series RLC Load2/LConn1 -- SG1/RConn1 -- Three-Phase Transformer (Two Windings)1/LConn1
  Three-Phase Series RLC Load2/LConn2 -- SG1/RConn2 -- Three-Phase Transformer (Two Windings)1/LConn2
  Three-Phase Series RLC Load2/LConn3 -- SG1/RConn3 -- Three-Phase Transformer (Two Windings)1/LConn3
  IBR2/RConn3 -- Three-Phase Transformer (Two Windings)5/LConn3
  B8_IBR2/LConn2 -- Three-Phase Transformer (Two Windings)5/RConn2
  B8_IBR2/LConn3 -- Three-Phase Transformer (Two Windings)5/RConn3
  B8_IBR2/LConn1 -- Three-Phase Transformer (Two Windings)5/RConn1
  IBR2/RConn2 -- Three-Phase Transformer (Two Windings)5/LConn2
  Ground4/LConn1 -- IBR2/LConn1
  IBR2/RConn1 -- Three-Phase Transformer (Two Windings)5/LConn1
  Three-Phase Transformer (Two Windings)1/RConn1 -- B1_SG1/LConn1
  Three-Phase Transformer (Two Windings)1/RConn2 -- B1_SG1/LConn2
  Three-Phase Transformer (Two Windings)1/RConn3 -- B1_SG1/LConn3
  Three-Phase Series RLC Load1/LConn1 -- Three-Phase Breaker/LConn1
  Three-Phase Series RLC Load1/LConn2 -- Three-Phase Breaker/LConn2
  Three-Phase Series RLC Load1/LConn3 -- Three-Phase Breaker/LConn3
  Three-Phase Transformer (Two Windings)6/LConn1 -- SG2/RConn1 -- Three-Phase Series RLC Load4/LConn1
  Three-Phase Series RLC Load4/LConn2 -- SG2/RConn2 -- Three-Phase Transformer (Two Windings)6/LConn2
  Three-Phase Series RLC Load4/LConn3 -- SG2/RConn3 -- Three-Phase Transformer (Two Windings)6/LConn3
  B9_SG2/LConn1 -- Three-Phase Transformer (Two Windings)6/RConn1
  B9_SG2/LConn2 -- Three-Phase Transformer (Two Windings)6/RConn2
  B9_SG2/LConn3 -- Three-Phase Transformer (Two Windings)6/RConn3
  B9_SG2/RConn1 -- B9_L/LConn1 -- TX1/LConn1 -- TX2/RConn1
  B9_SG2/RConn2 -- B9_L/LConn2 -- TX2/RConn2 -- TX1/LConn2
  B9_SG2/RConn3 -- B9_L/LConn3 -- TX1/LConn3 -- TX2/RConn3
  Three-Phase Series RLC Load5/LConn3 -- SG3/RConn3 -- Three-Phase Transformer (Two Windings)7/LConn3
  Three-Phase Series RLC Load5/LConn2 -- SG3/RConn2 -- Three-Phase Transformer (Two Windings)7/LConn2
  Three-Phase Transformer (Two Windings)7/LConn1 -- SG3/RConn1 -- Three-Phase Series RLC Load5/LConn1
  B8_SG3/LConn1 -- Three-Phase Transformer (Two Windings)7/RConn1
  B8_SG3/LConn3 -- Three-Phase Transformer (Two Windings)7/RConn3
  B8_SG3/LConn2 -- Three-Phase Transformer (Two Windings)7/RConn2
  Three-Phase Transformer (Two Windings)2/LConn1 -- IBR1/RConn1
  Three-Phase Transformer (Two Windings)2/LConn2 -- IBR1/RConn2
  IBR1/RConn3 -- Three-Phase Transformer (Two Windings)2/LConn3
  Three-Phase Transformer (Two Windings)2/RConn1 -- B1_IBR1/LConn1
  Three-Phase Transformer (Two Windings)2/RConn2 -- B1_IBR1/LConn2
  Three-Phase Transformer (Two Windings)2/RConn3 -- B1_IBR1/LConn3
  Ground1/LConn1 -- IBR1/LConn1
  B7_SG4/LConn1 -- Three-Phase Transformer (Two Windings)3/RConn1
  B7_SG4/LConn3 -- Three-Phase Transformer (Two Windings)3/RConn3
  B7_SG4/LConn2 -- Three-Phase Transformer (Two Windings)3/RConn2
  TX3/RConn1 -- TX4/LConn1 -- B7_IBR4/RConn1 -- B7_L/LConn1 -- B7_SG4/RConn1
  TX3/RConn2 -- TX4/LConn2 -- B7_IBR4/RConn2 -- B7_L/LConn2 -- B7_SG4/RConn2
  TX3/RConn3 -- B7_IBR4/RConn3 -- B7_L/LConn3 -- B7_SG4/RConn3 -- TX4/LConn3
  SG4/RConn1 -- Three-Phase Series RLC Load11/LConn1 -- Three-Phase Transformer (Two Windings)3/LConn1
  SG4/RConn2 -- Three-Phase Series RLC Load11/LConn2 -- Three-Phase Transformer (Two Windings)3/LConn2
  SG4/RConn3 -- Three-Phase Series RLC Load11/LConn3 -- Three-Phase Transformer (Two Windings)3/LConn3
  Three-Phase Series RLC Load3/LConn1 -- Three-Phase Breaker1/RConn1 -- B7_L/RConn1
  Three-Phase Series RLC Load3/LConn3 -- Three-Phase Breaker1/RConn3 -- B7_L/RConn3
  Three-Phase Series RLC Load3/LConn2 -- B7_L/RConn2 -- Three-Phase Breaker1/RConn2
  Three-Phase Series RLC Load6/LConn3 -- Three-Phase Breaker1/LConn3
  Three-Phase Series RLC Load6/LConn2 -- Three-Phase Breaker1/LConn2
  Three-Phase Series RLC Load6/LConn1 -- Three-Phase Breaker1/LConn1
  TX4/RConn2 -- Three-Phase Parallel RLC Load1/LConn2 -- B6_IBR3/RConn2 -- TX5/RConn2 -- B6_SG5/RConn2
  B6_SG5/LConn1 -- Three-Phase Transformer (Two Windings)4/RConn1
  B6_SG5/LConn2 -- Three-Phase Transformer (Two Windings)4/RConn2
  B6_SG5/LConn3 -- Three-Phase Transformer (Two Windings)4/RConn3
  SG5/RConn1 -- Three-Phase Series RLC Load7/LConn1 -- Three-Phase Transformer (Two Windings)4/LConn1
  SG5/RConn2 -- Three-Phase Series RLC Load7/LConn2 -- Three-Phase Transformer (Two Windings)4/LConn2
  SG5/RConn3 -- Three-Phase Series RLC Load7/LConn3 -- Three-Phase Transformer (Two Windings)4/LConn3
  Ground2/LConn1 -- IBR3/LConn1
  Three-Phase Transformer (Two Windings)8/LConn1 -- IBR3/RConn1
  Three-Phase Transformer (Two Windings)8/LConn2 -- IBR3/RConn2
  Three-Phase Transformer (Two Windings)8/LConn3 -- IBR3/RConn3
  Three-Phase Series RLC Load8/LConn2 -- SG6/RConn2 -- Three-Phase Transformer (Two Windings)9/LConn2
  Three-Phase Series RLC Load8/LConn1 -- SG6/RConn1 -- Three-Phase Transformer (Two Windings)9/LConn1
  Three-Phase Series RLC Load8/LConn3 -- SG6/RConn3 -- Three-Phase Transformer (Two Windings)9/LConn3
  B5_SG6/LConn2 -- Three-Phase Transformer (Two Windings)9/RConn2
  B5_SG6/LConn1 -- Three-Phase Transformer (Two Windings)9/RConn1
  B5_SG6/LConn3 -- Three-Phase Transformer (Two Windings)9/RConn3
  B5_L/LConn1 -- TX6/RConn1 -- TX5/LConn1 -- B5_SG6/RConn1
  TX6/RConn2 -- TX5/LConn2 -- B5_L/LConn2 -- B5_SG6/RConn2
  B5_L/LConn3 -- TX6/RConn3 -- TX5/LConn3 -- B5_SG6/RConn3
  Three-Phase Series RLC Load10/LConn2 -- Three-Phase Breaker2/LConn2
  Three-Phase Series RLC Load10/LConn3 -- Three-Phase Breaker2/LConn3
  Three-Phase Series RLC Load10/LConn1 -- Three-Phase Breaker2/LConn1
  TX4/RConn1 -- Three-Phase Parallel RLC Load1/LConn1 -- B6_IBR3/RConn1 -- TX5/RConn1 -- B6_SG5/RConn1
  TX4/RConn3 -- TX5/RConn3 -- Three-Phase Parallel RLC Load1/LConn3 -- B6_IBR3/RConn3 -- B6_SG5/RConn3
  B8_SG3/RConn1 -- B8_IBR2/RConn1 -- TX3/LConn1 -- TX2/LConn1
  B8_SG3/RConn2 -- B8_IBR2/RConn2 -- TX3/LConn2 -- TX2/LConn2
  B8_SG3/RConn3 -- B8_IBR2/RConn3 -- TX3/LConn3 -- TX2/LConn3
  B6_IBR3/LConn1 -- Three-Phase Transformer (Two Windings)8/RConn1
  B6_IBR3/LConn2 -- Three-Phase Transformer (Two Windings)8/RConn2
  B6_IBR3/LConn3 -- Three-Phase Transformer (Two Windings)8/RConn3
  TX1/RConn1 -- TX6/LConn1 -- B1_IBR1/RConn1 -- B1_SG1/RConn1
  TX1/RConn2 -- TX6/LConn2 -- B1_IBR1/RConn2 -- B1_SG1/RConn2
  TX1/RConn3 -- TX6/LConn3 -- B1_IBR1/RConn3 -- B1_SG1/RConn3
  Three-Phase Parallel RLC Load/LConn1 -- Three-Phase Breaker2/RConn1 -- B5_L/RConn1
  B5_L/RConn2 -- Three-Phase Breaker2/RConn2 -- Three-Phase Parallel RLC Load/LConn2
  Three-Phase Parallel RLC Load/LConn3 -- Three-Phase Breaker2/RConn3 -- B5_L/RConn3
  Three-Phase Parallel RLC Load2/LConn1 -- Three-Phase Breaker/RConn1 -- B9_L/RConn1
  Three-Phase Parallel RLC Load2/LConn2 -- B9_L/RConn2 -- Three-Phase Breaker/RConn2
  Three-Phase Parallel RLC Load2/LConn3 -- Three-Phase Breaker/RConn3 -- B9_L/RConn3
  B7_IBR4/LConn3 -- Three-Phase Transformer (Two Windings)10/RConn3
  IBR4/RConn3 -- Three-Phase Transformer (Two Windings)10/LConn3
  IBR4/RConn1 -- Three-Phase Transformer (Two Windings)10/LConn1
  IBR4/RConn2 -- Three-Phase Transformer (Two Windings)10/LConn2
  Ground3/LConn1 -- IBR4/LConn1
  B7_IBR4/LConn2 -- Three-Phase Transformer (Two Windings)10/RConn2
  B7_IBR4/LConn1 -- Three-Phase Transformer (Two Windings)10/RConn1
